simulink library "outp"  (R2021b)
(part 3 of 11)

  outpmodule/365(VOUTP_C3CCU1CSDTC_raw32) -> bus_creator/365
  bus_selector17/58 -> outpmodule/1117(VVMC_ADASWarningMsg_enum)  "<VVMC_ADASWarningMsg_enum>"
  bus_selector13/20 -> outpmodule/907(VTPM_RRWheelDebug_flg)  "<VTPM_RRWheelDebug_flg>"
  bus_selector17/62 -> outpmodule/1121(VVMC_LKAHODDisplayWarning_flg)  "<VVMC_LKAHODDisplayWarning_flg>"
  bus_selector17/53 -> outpmodule/1112(VVMC_ADASLDWSta_enum)  "<VVMC_ADASLDWSta_enum>"
  bus_selector17/50 -> outpmodule/1109(VVMC_RightTurnLightReq_flg)  "<VVMC_RightTurnLightReq_flg>"
  bus_selector17/47 -> outpmodule/1106(VVMC_ADASShftPosnReq_enum)  "<VVMC_ADASShftPosnReq_enum>"
  bus_selector17/46 -> outpmodule/1105(VVMC_ADASShftPosnReqA_flg)  "<VVMC_ADASShftPosnReqA_flg>"
  outpmodule/566(VOUTP_KeyAreaSPTGSta_enum) -> bus_creator/566
  bus_selector4/65 -> outpmodule/422(VDDM_FMLUSSDTC_raw32)  "<VDDM_FMLUSSDTC_raw32>"
  bus_selector9/3 -> outpmodule/611(VNMM_Awake_enum)  "<VNMM_Awake_enum>"
  outpmodule/81(VOUTP_RFPulseCount_enum) -> bus_creator/81
  outpmodule/479(VOUTP_RRWheelTmpHighDTC_raw32) -> bus_creator/479
  outpmodule/291(VOUTP_DimSwSta_flg) -> bus_creator/291
  bus_selector17/43 -> outpmodule/1102(VVMC_ACCJerkLowerLimit_mps3)  "<VVMC_ACCJerkLowerLimit_mps3>"
  bus_selector13/8 -> outpmodule/895(VTPM_RRWheelPress_raw8)  "<VTPM_RRWheelPress_raw8>"
  bus_selector2/60 -> outpmodule/63(VAPM_LFWhlRotDir_enum)  "<VAPM_LFWhlRotDir_enum>"
  bus_selector17/42 -> outpmodule/1101(VVMC_ACCComfortBandUpper_mps2)  "<VVMC_ACCComfortBandUpper_mps2>"
  outpmodule/551(VOUTP_PKELNumerator_kphsqr) -> bus_creator/551
  bus_selector7/47 -> outpmodule/601(VDKC_UWBDetArea_enum)  "<VDKC_UWBDetArea_enum>"
  bus_selector17/36 -> outpmodule/1095(VVMC_ADASDBSReq_enum)  "<VVMC_ADASDBSReq_enum>"
  bus_selector17/34 -> outpmodule/1093(VVMC_AEBVehHoldReq_flg)  "<VVMC_AEBVehHoldReq_flg>"
  bus_selector17/35 -> outpmodule/1094(VVMC_ACCVehHoldReq_flg)  "<VVMC_ACCVehHoldReq_flg>"
  bus_selector17/31 -> outpmodule/1090(VVMC_LKATOIAct_enum)  "<VVMC_LKATOIAct_enum>"
  outpmodule/556(VOUTP_DKCAuthSta_enum) -> bus_creator/556
  bus_selector17/32 -> outpmodule/1091(VVMC_ADASAEBReq_enum)  "<VVMC_ADASAEBReq_enum>"
  outpmodule/1063(VOUTP_MeterIndSpeed_raw32) -> bus_creator/1063
  bus_selector17/28 -> outpmodule/1087(VVMC_ADASLKASta_enum)  "<VVMC_ADASLKASta_enum>"
  bus_selector17/26 -> outpmodule/1085(VVMC_ActACCRequiredAccel_mps2)  "<VVMC_ActACCRequiredAccel_mps2>"
  bus_selector13/2 -> outpmodule/889(VTPM_RFBatWarn_flg)  "<VTPM_RFBatWarn_flg>"
  outpmodule/221(VOUTP_FrWiperL_flg) -> bus_creator/221
  bus_selector17/27 -> outpmodule/1086(VVMC_LateralCtrl_flg)  "<VVMC_LateralCtrl_flg>"
  bus_selector3/106 -> outpmodule/284(VBCM_AmbBrightnessSta1_enum)  "<VBCM_AmbBrightnessSta1_enum>"
  outpmodule/276(VOUTP_AmbPwrWarnENFlash_enum) -> bus_creator/276
  bus_selector2/38 -> outpmodule/41(VAPM_Chime_enum)  "<VAPM_Chime_enum>"
  bus_selector17/24 -> outpmodule/1083(VVMC_DISCReqAcc_mps2)  "<VVMC_DISCReqAcc_mps2>"
  bus_selector17/23 -> outpmodule/1082(VVMC_ACCRequiredAccel_mps2)  "<VVMC_ACCRequiredAccel_mps2>"
  bus_selector17/22 -> outpmodule/1081(VVMC_ISOJerkLimit_mps3)  "<VVMC_ISOJerkLimit_mps3>"
  bus_selector17/19 -> outpmodule/1078(VVMC_AccCalcuPID_mps2)  "<VVMC_AccCalcuPID_mps2>"
  outpmodule/450(VOUTP_ACCMalfuncDetDTC_raw32) -> bus_creator/450
  bus_selector17/18 -> outpmodule/1077(VVMC_SPD2ACCAct_flg)  "<VVMC_SPD2ACCAct_flg>"
  bus_selector12/17 -> outpmodule/728(VTHC_FDFrRiAPTCHeatPwrCmd_W)  "<VTHC_FDFrRiAPTCHeatPwrCmd_W>"
  outpmodule/1088(VOUTP_LKAStrToqReq_Nm) -> bus_creator/1088
  outpmodule/518(VOUTP_LowIdleAccPedal_flg) -> bus_creator/518
  outpmodule/909(VOUTP_TPMSCaliButtAllow_flg) -> bus_creator/909
  bus_selector7/48 -> outpmodule/602(VDKC_OutputPCMDModule_enum)  "<VDKC_OutputPCMDModule_enum>"
  outpmodule/415(VOUTP_EnterNewOperCyc_flg) -> bus_creator/415
  bus_selector12/16 -> outpmodule/727(VTHC_FDFrLeAPTCHeatPwrCmd_W)  "<VTHC_FDFrLeAPTCHeatPwrCmd_W>"
  bus_selector12/14 -> outpmodule/725(VTHC_FDEWP2Cmd_enum)  "<VTHC_FDEWP2Cmd_enum>"
  outpmodule/410(VOUTP_MCUR1NoComDTC_raw32) -> bus_creator/410
  bus_selector17/60 -> outpmodule/1119(VVMC_TargetType_enum)  "<VVMC_TargetType_enum>"
  outpmodule/278(VOUTP_AmbColorSta1_enum) -> bus_creator/278
  bus_selector12/15 -> outpmodule/726(VTHC_FDEWP3Cmd_enum)  "<VTHC_FDEWP3Cmd_enum>"
  bus_selector12/12 -> outpmodule/723(VTHC_FDAGSCmd_enum)  "<VTHC_FDAGSCmd_enum>"
  outpmodule/938(VOUTP_LFP20_raw8) -> bus_creator/938
  outpmodule/944(VOUTP_S1WheelDebugALTU_pct) -> bus_creator/944
  bus_selector12/13 -> outpmodule/724(VTHC_FDEWP1Cmd_enum)  "<VTHC_FDEWP1Cmd_enum>"
  bus_selector12/11 -> outpmodule/722(VTHC_CoolgFanActDuty_pct)  "<VTHC_CoolgFanActDuty_pct>"
  bus_selector12/9 -> outpmodule/720(VTHC_FDTWVCmd_pct)  "<VTHC_FDTWVCmd_pct>"
  outpmodule/137(VOUTP_AVMparkingcancel_enum) -> bus_creator/137
  outpmodule/929(VOUTP_S1ID_raw32) -> bus_creator/929
  bus_selector7/8 -> outpmodule/562(VDKC_KeyNumSta_enum)  "<VDKC_KeyNumSta_enum>"
  bus_selector3/43 -> outpmodule/221(VBCM_FrWiperL_flg)  "<VBCM_FrWiperL_flg>"
  outpmodule/886(VOUTP_FDCFGSFuncSta_flg) -> bus_creator/886
  bus_selector12/10 -> outpmodule/721(VTHC_FDFrWPTCHeatPwrCmd_W)  "<VTHC_FDFrWPTCHeatPwrCmd_W>"
  bus_selector12/6 -> outpmodule/717(VTHC_FDEXV2Cmd_step)  "<VTHC_FDEXV2Cmd_step>"
  outpmodule/100(VOUTP_SASCALTimeOut_flg) -> bus_creator/100
  bus_selector7/29 -> outpmodule/583(VDKC_UWBDetPTGArea_enum)  "<VDKC_UWBDetPTGArea_enum>"
  outpmodule/198(VOUTP_Dimmer_pct) -> bus_creator/198
  outpmodule/361(VOUTP_C3BMS1RCDTC_raw32) -> bus_creator/361
  outpmodule/223(VOUTP_RrWiper_flg) -> bus_creator/223
  bus_selector12/7 -> outpmodule/718(VTHC_FDSOTXVCmd_flg)  "<VTHC_FDSOTXVCmd_flg>"
  bus_selector17/2 -> outpmodule/1061(VVMC_VehicleSpeed_mph)  "<VVMC_VehicleSpeed_mph>"
  outpmodule/585(VOUTP_ParkingModeCmd_enum) -> bus_creator/585
  bus_selector2/100 -> outpmodule/103(VAPM_GRADE_Deg)  "<VAPM_GRADE_Deg>"
  bus_selector12/4 -> outpmodule/715(VTHC_FDSOV3Cmd_flg)  "<VTHC_FDSOV3Cmd_flg>"
  bus_selector12/2 -> outpmodule/713(VTHC_FDSOV1Cmd_flg)  "<VTHC_FDSOV1Cmd_flg>"
  bus_selector2/103 -> outpmodule/106(VAPM_YawRateTimeOut_flg)  "<VAPM_YawRateTimeOut_flg>"
  outpmodule/72(VOUTP_LFPulseCountVTimeOut_flg) -> bus_creator/72
  bus_selector12/97 -> outpmodule/808(VTHC_AirIntenZone3MSet7_enum)  "<VTHC_AirIntenZone3MSet7_enum>"
  bus_selector12/3 -> outpmodule/714(VTHC_FDSOV2Cmd_flg)  "<VTHC_FDSOV2Cmd_flg>"
  outpmodule/690(VOUTP_SHA1_cnt) -> bus_creator/690
  outpmodule/134(VOUTP_EPBErrStaTimeOut_flg) -> bus_creator/134
  bus_selector3/75 -> outpmodule/253(VBCM_MFRDNBrightReq_pct)  "<VBCM_MFRDNBrightReq_pct>"
  bus_selector11/17 -> outpmodule/685(VSYS_Variation_cnt)  "<VSYS_Variation_cnt>"
  bus_selector14/46 -> outpmodule/1030(VTQD_OPDHoldLamp_flg)  "<VTQD_OPDHoldLamp_flg>"
  bus_selector11/15 -> outpmodule/683(VSYS_Country1_cnt)  "<VSYS_Country1_cnt>"
  bus_selector7/12 -> outpmodule/566(VDKC_KeyAreaSPTGSta_enum)  "<VDKC_KeyAreaSPTGSta_enum>"
  bus_selector11/12 -> outpmodule/680(VSYS_Minor2_cnt)  "<VSYS_Minor2_cnt>"
  bus_selector13/9 -> outpmodule/896(VTPM_LFWheelTemp_C)  "<VTPM_LFWheelTemp_C>"
  outpmodule/629(VOUTP_HVSysReadyToCharge_enum) -> bus_creator/629
  bus_selector3/138 -> outpmodule/316(VBCM_WelcomeLight_enum)  "<VBCM_WelcomeLight_enum>"
  bus_selector11/10 -> outpmodule/678(VSYS_Major2_cnt)  "<VSYS_Major2_cnt>"
  outpmodule/774(VOUTP_FDCTHCCLVentENSta_flg) -> bus_creator/774
  bus_selector11/6 -> outpmodule/674(VSYS_CarModel3_cnt)  "<VSYS_CarModel3_cnt>"
  bus_selector11/5 -> outpmodule/673(VSYS_CarModel2_cnt)  "<VSYS_CarModel2_cnt>"
  outpmodule/215(VOUTP_MirrorDefog_flg) -> bus_creator/215
  outpmodule/315(VOUTP_HoodRelCmd_flg) -> bus_creator/315
  bus_selector17/49 -> outpmodule/1108(VVMC_HazardWarningReq_flg)  "<VVMC_HazardWarningReq_flg>"
  bus_selector11/3 -> outpmodule/671(VSYS_HWVer3_cnt)  "<VSYS_HWVer3_cnt>"
  outpmodule/1035(VOUTP_SetSpd_kph) -> bus_creator/1035
  bus_selector13/64 -> outpmodule/951(VTPM_ID4messageALTU_raw8)  "<VTPM_ID4messageALTU_raw8>"
  bus_selector12/18 -> outpmodule/729(VTHC_FDRrAPTCHeatPwrCmd_W)  "<VTHC_FDRrAPTCHeatPwrCmd_W>"
  outpmodule/1124(VOUTP_ADASLaneModeL_enum) -> bus_creator/1124
  bus_selector11/4 -> outpmodule/672(VSYS_CarModel1_cnt)  "<VSYS_CarModel1_cnt>"
  outpmodule/419(VOUTP_DiagRLTSDTC_raw32) -> bus_creator/419
  bus_selector11/1 -> outpmodule/669(VSYS_HWVer1_cnt)  "<VSYS_HWVer1_cnt>"
  BPMM_outputs/1 -> bus_selector10/1
  bus_selector10/47 -> outpmodule/667(VPMM_OTAPwrReqStdChkSta_enum)  "<VPMM_OTAPwrReqStdChkSta_enum>"
  outpmodule/115(VOUTP_LatAccelV_flg) -> bus_creator/115
  bus_selector13/41 -> outpmodule/928(VTPM_RRSensorMode_flg)  "<VTPM_RRSensorMode_flg>"
  outpmodule/839(VOUTP_FDCTHCREVentZStaSet7_enum) -> bus_creator/839
  bus_selector10/46 -> outpmodule/666(VPMM_OTAPwrReqOFFChkSta_enum)  "<VPMM_OTAPwrReqOFFChkSta_enum>"
  bus_selector3/123 -> outpmodule/301(VBCM_TurnSwTimeSetSta457_enum)  "<VBCM_TurnSwTimeSetSta457_enum>"
  bus_selector10/48 -> outpmodule/668(VPMM_PwrReqRAPSAvail_flg)  "<VPMM_PwrReqRAPSAvail_flg>"
  bus_selector12/105 -> outpmodule/816(VTHC_RVentENSet_enum)  "<VTHC_RVentENSet_enum>"
  bus_selector2/136 -> outpmodule/139(VAPM_AVMparkingexcute_enum)  "<VAPM_AVMparkingexcute_enum>"
  bus_selector10/44 -> outpmodule/664(VPMM_Sched_ChgTOSta_enum)  "<VPMM_Sched_ChgTOSta_enum>"
  bus_selector4/147 -> outpmodule/504(VDDM_SysAllowReadySta_flg)  "<VDDM_SysAllowReadySta_flg>"
  bus_selector7/26 -> outpmodule/580(VDKC_AllowSleep_flg)  "<VDKC_AllowSleep_flg>"
  bus_selector14/43 -> outpmodule/1027(VTQD_ActParkRequest_flg)  "<VTQD_ActParkRequest_flg>"
  bus_selector10/45 -> outpmodule/665(VPMM_PwrReq_OTA_enum)  "<VPMM_PwrReq_OTA_enum>"
  bus_selector3/30 -> outpmodule/208(VBCM_LBSD_flg)  "<VBCM_LBSD_flg>"
  bus_selector4/121 -> outpmodule/478(VDDM_LRWheelTmpHighDTC_raw32)  "<VDDM_LRWheelTmpHighDTC_raw32>"
  outpmodule/508(VOUTP_CAN2BusErrorDTC_raw32) -> bus_creator/508
  bus_selector12/69 -> outpmodule/780(VTHC_FDCFGSAirIntSta_enum)  "<VTHC_FDCFGSAirIntSta_enum>"
  bus_selector12/68 -> outpmodule/779(VTHC_FDCTHCMAPTCForceOFFSta_flg)  "<VTHC_FDCTHCMAPTCForceOFFSta_flg>"
  bus_selector1/1 -> outpmodule/1(VACC_HVTHCMSysAvail_enum)  "<VACC_HVTHCMSysAvail_enum>"
  bus_selector12/64 -> outpmodule/775(VTHC_FDCTHCREVentYSta_enum)  "<VTHC_FDCTHCREVentYSta_enum>"
  bus_selector12/67 -> outpmodule/778(VTHC_FDCTHCCRVentENSta_flg)  "<VTHC_FDCTHCCRVentENSta_flg>"
  outpmodule/120(VOUTP_MCPressureVTimeOut_flg) -> bus_creator/120
  outpmodule/238(VOUTP_AmbLightColor1_enum) -> bus_creator/238
  bus_selector12/65 -> outpmodule/776(VTHC_FDCTHCRVentENSta_flg)  "<VTHC_FDCTHCRVentENSta_flg>"
  outpmodule/93(VOUTP_SASAngle_Deg) -> bus_creator/93
  bus_selector12/62 -> outpmodule/773(VTHC_FDCTHCCLEVentYSta_enum)  "<VTHC_FDCTHCCLEVentYSta_enum>"
  bus_selector12/61 -> outpmodule/772(VTHC_FDCTHCLVentENSta_flg)  "<VTHC_FDCTHCLVentENSta_flg>"
  bus_selector12/60 -> outpmodule/771(VTHC_FDCTHCLEVentYSta_enum)  "<VTHC_FDCTHCLEVentYSta_enum>"
  outpmodule/454(VOUTP_MCUF1RCErrDTC_raw32) -> bus_creator/454
  outpmodule/874(VOUTP_SettempZon1Set5_enum) -> bus_creator/874
  outpmodule/888(VOUTP_LFBatWarn_flg) -> bus_creator/888
  bus_selector12/59 -> outpmodule/770(VTHC_FDCTHCCREVentZSta_enum)  "<VTHC_FDCTHCCREVentZSta_enum>"
  bus_selector2/51 -> outpmodule/54(VAPM_RRRawWhlSpeedTimeOut_flg)  "<VAPM_RRRawWhlSpeedTimeOut_flg>"
  bus_selector12/55 -> outpmodule/766(VTHC_FDCTHCREVentModeSta_enum)  "<VTHC_FDCTHCREVentModeSta_enum>"
  bus_selector12/57 -> outpmodule/768(VTHC_FDCTHCCLEVentZSta_enum)  "<VTHC_FDCTHCCLEVentZSta_enum>"
  outpmodule/659(VOUTP_CtrlFrBMSCCUCIR_flg) -> bus_creator/659
  bus_selector12/53 -> outpmodule/764(VTHC_FDCTHCAirIntZ3Sta_enum)  "<VTHC_FDCTHCAirIntZ3Sta_enum>"
  bus_selector4/59 -> outpmodule/416(VDDM_DiagHCrashDTC_raw32)  "<VDDM_DiagHCrashDTC_raw32>"
  BACC_outputs/1 -> bus_selector1/1
  outpmodule/90(VOUTP_DriIntendTimeOut_flg) -> bus_creator/90
  bus_selector7/40 -> outpmodule/594(VDKC_BLERSSI_enum)  "<VDKC_BLERSSI_enum>"
  bus_selector12/52 -> outpmodule/763(VTHC_sigDfrstSt_flg)  "<VTHC_sigDfrstSt_flg>"
  bus_selector12/50 -> outpmodule/761(VTHC_fdefog_flg)  "<VTHC_fdefog_flg>"
  bus_selector12/48 -> outpmodule/759(VTHC_RecAutoFlg_flg)  "<VTHC_RecAutoFlg_flg>"
  bus_selector2/22 -> outpmodule/25(VAPM_PASARCL_enum)  "<VAPM_PASARCL_enum>"
  bus_selector11/2 -> outpmodule/670(VSYS_HWVer2_cnt)  "<VSYS_HWVer2_cnt>"
  outpmodule/122(VOUTP_BrkSwStaTimeOut_flg) -> bus_creator/122
  bus_selector12/46 -> outpmodule/757(VTHC_CCUSyncSts_flg)  "<VTHC_CCUSyncSts_flg>"
  outpmodule/126(VOUTP_ESCStandstillTimeOut_flg) -> bus_creator/126
  outpmodule/882(VOUTP_CLVentEN_flg) -> bus_creator/882
  bus_selector9/5 -> outpmodule/613(VNMM_ErrorState_enum)  "<VNMM_ErrorState_enum>"
  outpmodule/214(VOUTP_MirrorCtrl_enum) -> bus_creator/214
  outpmodule/577(VOUTP_FDCSPTGOpen_flg) -> bus_creator/577
  bus_selector2/82 -> outpmodule/85(VAPM_RRPulseCount_enum)  "<VAPM_RRPulseCount_enum>"
  bus_selector3/2 -> outpmodule/180(VBCM_TailgateRemote_enum)  "<VBCM_TailgateRemote_enum>"
  outpmodule/1171(VOUTP_FDCVMCAPSRqEPSCtrl_flg) -> bus_creator/1171
  bus_selector12/63 -> outpmodule/774(VTHC_FDCTHCCLVentENSta_flg)  "<VTHC_FDCTHCCLVentENSta_flg>"
  bus_selector12/44 -> outpmodule/755(VTHC_FaceM_flg)  "<VTHC_FaceM_flg>"
  outpmodule/11(VOUTP_PASDRCR_cm) -> bus_creator/11
  bus_selector12/45 -> outpmodule/756(VTHC_FootM_flg)  "<VTHC_FootM_flg>"
  outpmodule/128(VOUTP_ESCAPSStaTimeOut_flg) -> bus_creator/128
  bus_selector2/104 -> outpmodule/107(VAPM_LatAccel_Gps)  "<VAPM_LatAccel_Gps>"
  bus_selector12/42 -> outpmodule/753(VTHC_Foot_flg)  "<VTHC_Foot_flg>"
  bus_selector2/144 -> outpmodule/147(VAPM_CAASSw_enum)  "<VAPM_CAASSw_enum>"
  outpmodule/780(VOUTP_FDCFGSAirIntSta_enum) -> bus_creator/780
  outpmodule/530(VOUTP_APPD_pct) -> bus_creator/530
  bus_selector7/35 -> outpmodule/589(VDKC_DKeyWelcomeSta_enum)  "<VDKC_DKeyWelcomeSta_enum>"
  bus_selector12/39 -> outpmodule/750(VTHC_FDRecyAutoCmd_enum)  "<VTHC_FDRecyAutoCmd_enum>"
  bus_selector2/93 -> outpmodule/96(VAPM_SASSpeedTimeOut_flg)  "<VAPM_SASSpeedTimeOut_flg>"
  outpmodule/96(VOUTP_SASSpeedTimeOut_flg) -> bus_creator/96
  bus_selector12/43 -> outpmodule/754(VTHC_Frost_flg)  "<VTHC_Frost_flg>"
  outpmodule/707(VOUTP_PmicBootPath_raw32) -> bus_creator/707
  bus_selector17/63 -> outpmodule/1122(VVMC_LKAHODSoundWarning_flg)  "<VVMC_LKAHODSoundWarning_flg>"
  bus_selector2/16 -> outpmodule/19(VAPM_APSDFLR_cm)  "<VAPM_APSDFLR_cm>"
  bus_selector12/41 -> outpmodule/752(VTHC_Face_flg)  "<VTHC_Face_flg>"
  bus_selector2/156 -> outpmodule/159(VAPM_APSSWVer_enum)  "<VAPM_APSSWVer_enum>"
  bus_selector12/34 -> outpmodule/745(VTHC_sigClntTHvBattIn_C)  "<VTHC_sigClntTHvBattIn_C>"
  bus_selector12/36 -> outpmodule/747(VTHC_sigAmbAirT_C)  "<VTHC_sigAmbAirT_C>"
  bus_selector17/21 -> outpmodule/1080(VVMC_ISODecLimit_mps2)  "<VVMC_ISODecLimit_mps2>"
  bus_selector11/8 -> outpmodule/676(VSYS_ECU2_cnt)  "<VSYS_ECU2_cnt>"
  bus_selector12/33 -> outpmodule/744(VTHC_sigCbnSolarLeft_W)  "<VTHC_sigCbnSolarLeft_W>"
  bus_selector12/32 -> outpmodule/743(VTHC_sigClntTHvBattOut_C)  "<VTHC_sigClntTHvBattOut_C>"
  outpmodule/294(VOUTP_FWasSwSta_enum) -> bus_creator/294
  outpmodule/83(VOUTP_LRPulseCount_enum) -> bus_creator/83
  bus_selector12/29 -> outpmodule/740(VTHC_sigRecircSt_flg)  "<VTHC_sigRecircSt_flg>"
  bus_selector12/31 -> outpmodule/742(VTHC_sigSetTempZon2St_C)  "<VTHC_sigSetTempZon2St_C>"
  bus_selector12/28 -> outpmodule/739(VTHC_sigWindDirZon1St_enum)  "<VTHC_sigWindDirZon1St_enum>"
  bus_selector3/98 -> outpmodule/276(VBCM_AmbPwrWarnENFlash_enum)  "<VBCM_AmbPwrWarnENFlash_enum>"
  bus_selector17/105 -> outpmodule/1164(VVMC_CalibratedAccY_G)  "<VVMC_CalibratedAccY_G>"
  bus_selector4/23 -> outpmodule/380(VDDM_ONtoRdyDTC_raw32)  "<VDDM_ONtoRdyDTC_raw32>"
  bus_selector10/29 -> outpmodule/649(VPMM_LVBattChrgTimeCnt_s)  "<VPMM_LVBattChrgTimeCnt_s>"
  outpmodule/108(VOUTP_LatAccelTimeOut_flg) -> bus_creator/108
  bus_selector12/27 -> outpmodule/738(VTHC_sigAirIntenZon1St_enum)  "<VTHC_sigAirIntenZon1St_enum>"
  bus_selector3/57 -> outpmodule/235(VBCM_AmbLightBrightness4_enum)  "<VBCM_AmbLightBrightness4_enum>"
  outpmodule/919(VOUTP_LFWheelPSW_raw8) -> bus_creator/919
  bus_selector13/32 -> outpmodule/919(VTPM_LFWheelPSW_raw8)  "<VTPM_LFWheelPSW_raw8>"
  outpmodule/734(VOUTP_CCUACLampSts_flg) -> bus_creator/734
  bus_selector12/25 -> outpmodule/736(VTHC_CCUACMaxLampSts_flg)  "<VTHC_CCUACMaxLampSts_flg>"
  bus_selector12/22 -> outpmodule/733(VTHC_CabinMode_enum)  "<VTHC_CabinMode_enum>"
  outpmodule/412(VOUTP_ESC7NoComDTC_raw32) -> bus_creator/412
  bus_selector12/167 -> outpmodule/878(VTHC_FACESet_enum)  "<VTHC_FACESet_enum>"
  bus_selector12/166 -> outpmodule/877(VTHC_ACModeSet457_enum)  "<VTHC_ACModeSet457_enum>"
  outpmodule/935(VOUTP_S3L_enum) -> bus_creator/935
  bus_selector4/41 -> outpmodule/398(VDDM_FLDoorSWDTC_raw32)  "<VDDM_FLDoorSWDTC_raw32>"
  bus_selector12/168 -> outpmodule/879(VTHC_FOOTSet_enum)  "<VTHC_FOOTSet_enum>"
  bus_selector12/164 -> outpmodule/875(VTHC_SettempZon1Set7_enum)  "<VTHC_SettempZon1Set7_enum>"
  bus_selector4/9 -> outpmodule/366(VDDM_C3CCU1LCDTC_raw32)  "<VDDM_C3CCU1LCDTC_raw32>"
  bus_selector12/8 -> outpmodule/719(VTHC_FDFWVCmd_flg)  "<VTHC_FDFWVCmd_flg>"
  bus_selector17/48 -> outpmodule/1107(VVMC_ADASForceIdle_flg)  "<VVMC_ADASForceIdle_flg>"
  bus_selector17/29 -> outpmodule/1088(VVMC_LKAStrToqReq_Nm)  "<VVMC_LKAStrToqReq_Nm>"
  outpmodule/590(VOUTP_UWB1Distance_enum) -> bus_creator/590
  bus_selector12/162 -> outpmodule/873(VTHC_SettempZon1Set4_enum)  "<VTHC_SettempZon1Set4_enum>"
  bus_selector12/163 -> outpmodule/874(VTHC_SettempZon1Set5_enum)  "<VTHC_SettempZon1Set5_enum>"
  bus_selector17/38 -> outpmodule/1097(VVMC_ACCObjDist_m)  "<VVMC_ACCObjDist_m>"
  bus_selector7/38 -> outpmodule/592(VDKC_UWB3Distance_enum)  "<VDKC_UWB3Distance_enum>"
  bus_selector12/161 -> outpmodule/872(VTHC_SettempZon1Set3_enum)  "<VTHC_SettempZon1Set3_enum>"
  bus_selector12/159 -> outpmodule/870(VTHC_SettempZon1Set1_enum)  "<VTHC_SettempZon1Set1_enum>"
  outpmodule/738(VOUTP_sigAirIntenZon1St_enum) -> bus_creator/738
  bus_selector17/65 -> outpmodule/1124(VVMC_ADASLaneModeL_enum)  "<VVMC_ADASLaneModeL_enum>"
  bus_selector12/158 -> outpmodule/869(VTHC_FDCTHCCREVentYStaSet7_enum)  "<VTHC_FDCTHCCREVentYStaSet7_enum>"
  outpmodule/1163(VOUTP_CalibratedAccX_G) -> bus_creator/1163
  bus_selector3/24 -> outpmodule/202(VBCM_HBeam_flg)  "<VBCM_HBeam_flg>"
  bus_selector13/37 -> outpmodule/924(VTPM_AutoLTips_enum)  "<VTPM_AutoLTips_enum>"
  bus_selector17/37 -> outpmodule/1096(VVMC_ADASACCSta_enum)  "<VVMC_ADASACCSta_enum>"
  bus_selector12/155 -> outpmodule/866(VTHC_FDCTHCCREVentYStaSet3_enum)  "<VTHC_FDCTHCCREVentYStaSet3_enum>"
  bus_selector3/69 -> outpmodule/247(VBCM_FollowMe_flg)  "<VBCM_FollowMe_flg>"
  outpmodule/601(VOUTP_UWBDetArea_enum) -> bus_creator/601
  outpmodule/49(VOUTP_RFRawWhlSpeed_kph) -> bus_creator/49
  bus_selector12/151 -> outpmodule/862(VTHC_FDCTHCREVentYStaSet5_enum)  "<VTHC_FDCTHCREVentYStaSet5_enum>"
  bus_selector13/44 -> outpmodule/931(VTPM_S3ID_raw32)  "<VTPM_S3ID_raw32>"
  bus_selector4/18 -> outpmodule/375(VDDM_Lv3ErrDTC_raw32)  "<VDDM_Lv3ErrDTC_raw32>"
  outpmodule/438(VOUTP_FCM3CSErrDTC_raw32) -> bus_creator/438
  bus_selector17/40 -> outpmodule/1099(VVMC_TimeGapLevel_enum)  "<VVMC_TimeGapLevel_enum>"
  bus_selector12/153 -> outpmodule/864(VTHC_FDCTHCCREVentYStaSet1_enum)  "<VTHC_FDCTHCCREVentYStaSet1_enum>"
  outpmodule/51(VOUTP_LRRawWhlSpeed_kph) -> bus_creator/51
  bus_selector13/4 -> outpmodule/891(VTPM_RRBatWarn_flg)  "<VTPM_RRBatWarn_flg>"
  bus_selector4/53 -> outpmodule/410(VDDM_MCUR1NoComDTC_raw32)  "<VDDM_MCUR1NoComDTC_raw32>"
  outpmodule/655(VOUTP_LVSilentChrgReq_flg) -> bus_creator/655
  bus_selector12/154 -> outpmodule/865(VTHC_FDCTHCCREVentYStaSet2_enum)  "<VTHC_FDCTHCCREVentYStaSet2_enum>"
  bus_selector10/27 -> outpmodule/647(VPMM_IVIPwrStaONTOPopT_s)  "<VPMM_IVIPwrStaONTOPopT_s>"
  bus_selector12/149 -> outpmodule/860(VTHC_FDCTHCREVentYStaSet3_enum)  "<VTHC_FDCTHCREVentYStaSet3_enum>"
  bus_selector11/13 -> outpmodule/681(VSYS_Patch1_cnt)  "<VSYS_Patch1_cnt>"
  bus_selector4/83 -> outpmodule/440(VDDM_FCM4CSErrDTC_raw32)  "<VDDM_FCM4CSErrDTC_raw32>"
  outpmodule/453(VOUTP_ISAMalfuncDetDTC_raw32) -> bus_creator/453
  bus_selector12/150 -> outpmodule/861(VTHC_FDCTHCREVentYStaSet4_enum)  "<VTHC_FDCTHCREVentYStaSet4_enum>"
  outpmodule/300(VOUTP_TurnSwTimeSetSta123_enum) -> bus_creator/300
  bus_selector12/54 -> outpmodule/765(VTHC_FDCTHCLEVentModeSta_enum)  "<VTHC_FDCTHCLEVentModeSta_enum>"
  bus_selector12/146 -> outpmodule/857(VTHC_FDCTHCCLEVentYStaSet7_enum)  "<VTHC_FDCTHCCLEVentYStaSet7_enum>"
  bus_selector12/148 -> outpmodule/859(VTHC_FDCTHCREVentYStaSet2_enum)  "<VTHC_FDCTHCREVentYStaSet2_enum>"
  outpmodule/705(VOUTP_ECUGen1_cnt) -> bus_creator/705
  outpmodule/1045(VOUTP_FrTMTqReq_Nm) -> bus_creator/1045
  bus_selector17/41 -> outpmodule/1100(VVMC_ACCJerkUpperLimit_mps3)  "<VVMC_ACCJerkUpperLimit_mps3>"
  bus_selector12/147 -> outpmodule/858(VTHC_FDCTHCREVentYStaSet1_enum)  "<VTHC_FDCTHCREVentYStaSet1_enum>"
  bus_selector12/143 -> outpmodule/854(VTHC_FDCTHCCLEVentYStaSet3_enum)  "<VTHC_FDCTHCCLEVentYStaSet3_enum>"
  bus_selector4/72 -> outpmodule/429(VDDM_FLLUSSDTC_raw32)  "<VDDM_FLLUSSDTC_raw32>"
  bus_selector12/145 -> outpmodule/856(VTHC_FDCTHCCLEVentYStaSet5_enum)  "<VTHC_FDCTHCCLEVentYStaSet5_enum>"
  bus_selector12/141 -> outpmodule/852(VTHC_FDCTHCCLEVentYStaSet1_enum)  "<VTHC_FDCTHCCLEVentYStaSet1_enum>"
  bus_selector6/3 -> outpmodule/528(VDID_MILDIST_km)  "<VDID_MILDIST_km>"
  bus_selector11/11 -> outpmodule/679(VSYS_Minor1_cnt)  "<VSYS_Minor1_cnt>"
  outpmodule/1103(VOUTP_ACCComfortBandLower_mps2) -> bus_creator/1103
  bus_selector12/138 -> outpmodule/849(VTHC_FDCTHCLEVentYStaSet4_enum)  "<VTHC_FDCTHCLEVentYStaSet4_enum>"
  bus_selector17/52 -> outpmodule/1111(VVMC_ADASFCWSta_enum)  "<VVMC_ADASFCWSta_enum>"
  outpmodule/550(VOUTP_PKERNumerator_kphsqr) -> bus_creator/550
  bus_selector17/57 -> outpmodule/1116(VVMC_ACCTakeoverReq_flg)  "<VVMC_ACCTakeoverReq_flg>"
  bus_selector13/77 -> outpmodule/964(VTPM_WriteChkRRID_raw)  "<VTPM_WriteChkRRID_raw>"
  bus_selector4/81 -> outpmodule/438(VDDM_FCM3CSErrDTC_raw32)  "<VDDM_FCM3CSErrDTC_raw32>"
  bus_selector2/168 -> outpmodule/171(VAPM_APSSpeedCMD_kph)  "<VAPM_APSSpeedCMD_kph>"
  bus_selector9/4 -> outpmodule/612(VNMM_CSB_flg)  "<VNMM_CSB_flg>"
  bus_selector12/139 -> outpmodule/850(VTHC_FDCTHCLEVentYStaSet5_enum)  "<VTHC_FDCTHCLEVentYStaSet5_enum>"
  bus_selector4/156 -> outpmodule/513(VDDM_FrMCU4PreDTC_raw32)  "<VDDM_FrMCU4PreDTC_raw32>"
  outpmodule/686(VOUTP_Dash1_cnt) -> bus_creator/686
  outpmodule/287(VOUTP_AmbBrightnessSta4_enum) -> bus_creator/287
  bus_selector7/24 -> outpmodule/578(VDKC_UIDLowPowerSta_flg)  "<VDKC_UIDLowPowerSta_flg>"
  bus_selector2/3 -> outpmodule/6(VAPM_FSOffSw_enum)  "<VAPM_FSOffSw_enum>"
  bus_selector12/135 -> outpmodule/846(VTHC_FDCTHCLEVentYStaSet1_enum)  "<VTHC_FDCTHCLEVentYStaSet1_enum>"
  bus_selector3/97 -> outpmodule/275(VBCM_AmbLinkDriStaFlash_enum)  "<VBCM_AmbLinkDriStaFlash_enum>"
  bus_selector12/137 -> outpmodule/848(VTHC_FDCTHCLEVentYStaSet3_enum)  "<VTHC_FDCTHCLEVentYStaSet3_enum>"
  outpmodule/94(VOUTP_SASAngleTimeOut_flg) -> bus_creator/94
  outpmodule/505(VOUTP_VCUHoodSWSta_flg) -> bus_creator/505
  bus_selector13/52 -> outpmodule/939(VTPM_RFP20_raw8)  "<VTPM_RFP20_raw8>"
  outpmodule/670(VOUTP_HWVer2_cnt) -> bus_creator/670
  bus_selector17/55 -> outpmodule/1114(VVMC_ACCObjDstLvl_enum)  "<VVMC_ACCObjDstLvl_enum>"
  outpmodule/360(VOUTP_C3BMS6LCDTC_raw32) -> bus_creator/360
  bus_selector12/136 -> outpmodule/847(VTHC_FDCTHCLEVentYStaSet2_enum)  "<VTHC_FDCTHCLEVentYStaSet2_enum>"
  outpmodule/703(VOUTP_AcoreRebootCmdACK_flg) -> bus_creator/703
  bus_selector12/132 -> outpmodule/843(VTHC_FDCTHCCREVentZStaSet4_enum)  "<VTHC_FDCTHCCREVentZStaSet4_enum>"
  bus_selector7/15 -> outpmodule/569(VDKC_UWBOnOff_flg)  "<VDKC_UWBOnOff_flg>"
  outpmodule/538(VOUTP_CPSAR_sec) -> bus_creator/538
  bus_selector17/44 -> outpmodule/1103(VVMC_ACCComfortBandLower_mps2)  "<VVMC_ACCComfortBandLower_mps2>"
  bus_selector4/29 -> outpmodule/386(VDDM_DCDCEnaDTC_raw32)  "<VDDM_DCDCEnaDTC_raw32>"
  bus_selector7/36 -> outpmodule/590(VDKC_UWB1Distance_enum)  "<VDKC_UWB1Distance_enum>"
  outpmodule/404(VOUTP_EDriveSysErrVCUErr_flg) -> bus_creator/404
  outpmodule/644(VOUTP_ReVehThdChkSta_enum) -> bus_creator/644
  bus_selector3/99 -> outpmodule/277(VBCM_AmbODAENFlash_enum)  "<VBCM_AmbODAENFlash_enum>"
  bus_selector10/11 -> outpmodule/631(VPMM_LVPwrSta_flg)  "<VPMM_LVPwrSta_flg>"
  bus_selector2/4 -> outpmodule/7(VAPM_FSOffSwTimeOut_flg)  "<VAPM_FSOffSwTimeOut_flg>"
  bus_selector12/131 -> outpmodule/842(VTHC_FDCTHCCREVentZStaSet3_enum)  "<VTHC_FDCTHCCREVentZStaSet3_enum>"
  bus_selector12/129 -> outpmodule/840(VTHC_FDCTHCCREVentZStaSet1_enum)  "<VTHC_FDCTHCCREVentZStaSet1_enum>"
  BAPM_outputs/1 -> bus_selector2/1
  bus_selector7/50 -> outpmodule/604(VDKC_JudgeKeepUnlockZone_flg)  "<VDKC_JudgeKeepUnlockZone_flg>"
  outpmodule/1066(VOUTP_VMCCCCtrlAvail_flg) -> bus_creator/1066
  bus_selector3/80 -> outpmodule/258(VBCM_PsRWdwCtrlCmd_pct)  "<VBCM_PsRWdwCtrlCmd_pct>"
  bus_selector12/127 -> outpmodule/838(VTHC_FDCTHCREVentZStaSet5_enum)  "<VTHC_FDCTHCREVentZStaSet5_enum>"
  bus_selector12/128 -> outpmodule/839(VTHC_FDCTHCREVentZStaSet7_enum)  "<VTHC_FDCTHCREVentZStaSet7_enum>"
  outpmodule/835(VOUTP_FDCTHCREVentZStaSet2_enum) -> bus_creator/835
  outpmodule/1166(VOUTP_CalibratedGyroX_Dps) -> bus_creator/1166
  bus_selector17/54 -> outpmodule/1113(VVMC_ADASFltWrnReq_flg)  "<VVMC_ADASFltWrnReq_flg>"
  bus_selector12/126 -> outpmodule/837(VTHC_FDCTHCREVentZStaSet4_enum)  "<VTHC_FDCTHCREVentZStaSet4_enum>"
  bus_selector4/127 -> outpmodule/484(VDDM_C1EPAS2LCDTC_raw32)  "<VDDM_C1EPAS2LCDTC_raw32>"
  bus_selector12/123 -> outpmodule/834(VTHC_FDCTHCREVentZStaSet1_enum)  "<VTHC_FDCTHCREVentZStaSet1_enum>"
  bus_selector17/61 -> outpmodule/1120(VVMC_ADASSLIFSpdLim_enum)  "<VVMC_ADASSLIFSpdLim_enum>"
  bus_selector7/33 -> outpmodule/587(VDKC_ReVehData_enum)  "<VDKC_ReVehData_enum>"
  bus_selector4/66 -> outpmodule/423(VDDM_FMRUSSDTC_raw32)  "<VDDM_FMRUSSDTC_raw32>"
  bus_selector12/121 -> outpmodule/832(VTHC_FDCTHCCLEVentZStaSet5_enum)  "<VTHC_FDCTHCCLEVentZStaSet5_enum>"
  bus_selector12/124 -> outpmodule/835(VTHC_FDCTHCREVentZStaSet2_enum)  "<VTHC_FDCTHCREVentZStaSet2_enum>"
  bus_selector17/45 -> outpmodule/1104(VVMC_ADASVehSpdLim_raw32)  "<VVMC_ADASVehSpdLim_raw32>"
  bus_selector12/125 -> outpmodule/836(VTHC_FDCTHCREVentZStaSet3_enum)  "<VTHC_FDCTHCREVentZStaSet3_enum>"
  outpmodule/4(VOUTP_VehSpeed_kph) -> bus_creator/4
  outpmodule/484(VOUTP_C1EPAS2LCDTC_raw32) -> bus_creator/484
  outpmodule/3(VOUTP_VehHVPwrAvail4THCM_W) -> bus_creator/3
  bus_selector12/47 -> outpmodule/758(VTHC_ACForceOFF_flg)  "<VTHC_ACForceOFF_flg>"
  outpmodule/2(VOUTP_LVBattVoltSta_enum) -> bus_creator/2
  outpmodule/751(VOUTP_ACModeMem_enum) -> bus_creator/751
  bus_selector3/38 -> outpmodule/216(VBCM_RrDefog_flg)  "<VBCM_RrDefog_flg>"
  outpmodule/142(VOUTP_AVMParkingmodeTimeOut_flg) -> bus_creator/142
  outpmodule/1(VOUTP_HVTHCMSysAvail_enum) -> bus_creator/1
  outpmodule/740(VOUTP_sigRecircSt_flg) -> bus_creator/740
  outpmodule/516(VOUTP_RegenErrDTC_raw32) -> bus_creator/516
  outpmodule/371(VOUTP_C1ABM1CSDTC_raw32) -> bus_creator/371
  outpmodule/311(VOUTP_WalkInUnLkENFunSta_flg) -> bus_creator/311
  outpmodule/853(VOUTP_FDCTHCCLEVentYStaSet2_enum) -> bus_creator/853
  outpmodule/1100(VOUTP_ACCJerkUpperLimit_mps3) -> bus_creator/1100
  outpmodule/373(VOUTP_Lv1ErrDTC_raw32) -> bus_creator/373
  bus_selector4/87 -> outpmodule/444(VDDM_BMSSigErrDetDTC_raw32)  "<VDDM_BMSSigErrDetDTC_raw32>"
  outpmodule/353(VOUTP_CLWinLockDrStaMem_enum) -> bus_creator/353
  bus_selector4/11 -> outpmodule/368(VDDM_C3CCU2CSDTC_raw32)  "<VDDM_C3CCU2CSDTC_raw32>"
  outpmodule/1065(VOUTP_VMCACCCtrlAvail_flg) -> bus_creator/1065
  outpmodule/350(VOUTP_DrRWdwReqAP_enum) -> bus_creator/350
  outpmodule/352(VOUTP_CLWinLockDrSta_flg) -> bus_creator/352
  bus_selector13/82 -> outpmodule/969(VTPM_Flashchkdatavalid_enum)  "<VTPM_Flashchkdatavalid_enum>"
  bus_selector4/19 -> outpmodule/376(VDDM_Lv4ErrDTC_raw32)  "<VDDM_Lv4ErrDTC_raw32>"
  bus_selector3/36 -> outpmodule/214(VBCM_MirrorCtrl_enum)  "<VBCM_MirrorCtrl_enum>"
  outpmodule/349(VOUTP_PasWdwReqAP_enum) -> bus_creator/349
  bus_selector3/132 -> outpmodule/310(VBCM_FollowMeENMem_enum)  "<VBCM_FollowMeENMem_enum>"
  BNMM_outputs/1 -> bus_selector9/1
  outpmodule/801(VOUTP_AirIntenZone1MSet5_enum) -> bus_creator/801
  outpmodule/346(VOUTP_HMIKey8FuncSta_enum) -> bus_creator/346
  outpmodule/347(VOUTP_AutoWipHSpdENSta_flg) -> bus_creator/347
  bus_selector3/67 -> outpmodule/245(VBCM_SPTGDet_flg)  "<VBCM_SPTGDet_flg>"
  outpmodule/345(VOUTP_HMIKey7FuncSta_enum) -> bus_creator/345
  bus_selector2/15 -> outpmodule/18(VAPM_APSDRLL_cm)  "<VAPM_APSDRLL_cm>"
  outpmodule/341(VOUTP_HMIKey3FuncSta_enum) -> bus_creator/341
  outpmodule/87(VOUTP_ShifterHandleCmd_enum) -> bus_creator/87
  outpmodule/880(VOUTP_FrostSet_enum) -> bus_creator/880
  outpmodule/342(VOUTP_HMIKey4FuncSta_enum) -> bus_creator/342
  bus_selector12/51 -> outpmodule/762(VTHC_sigSetTempZon2StM_C)  "<VTHC_sigSetTempZon2StM_C>"
  bus_selector3/56 -> outpmodule/234(VBCM_AmbLightBrightness3_enum)  "<VBCM_AmbLightBrightness3_enum>"
  bus_selector3/21 -> outpmodule/199(VBCM_DimmerEN_flg)  "<VBCM_DimmerEN_flg>"
  bus_selector4/151 -> outpmodule/508(VDDM_CAN2BusErrorDTC_raw32)  "<VDDM_CAN2BusErrorDTC_raw32>"
  outpmodule/727(VOUTP_FDFrLeAPTCHeatPwrCmd_W) -> bus_creator/727
  outpmodule/368(VOUTP_C3CCU2CSDTC_raw32) -> bus_creator/368
  bus_selector12/70 -> outpmodule/781(VTHC_FDCFGSChSta_enum)  "<VTHC_FDCFGSChSta_enum>"
  outpmodule/537(VOUTP_IPSAL_sec) -> bus_creator/537
  outpmodule/363(VOUTP_C3BMS1LCDTC_raw32) -> bus_creator/363
  outpmodule/951(VOUTP_ID4messageALTU_raw8) -> bus_creator/951
  outpmodule/261(VOUTP_AmbWelEN_flg) -> bus_creator/261
  outpmodule/262(VOUTP_AmbDimEN_flg) -> bus_creator/262
  bus_selector4/47 -> outpmodule/404(VDDM_EDriveSysErrVCUErr_flg)  "<VDDM_EDriveSysErrVCUErr_flg>"
  bus_selector2/158 -> outpmodule/161(VAPM_APSExitCondition_enum)  "<VAPM_APSExitCondition_enum>"
  outpmodule/260(VOUTP_AmbFunEN_flg) -> bus_creator/260
  outpmodule/307(VOUTP_WalkOutLkENMem_enum) -> bus_creator/307
  outpmodule/546(VOUTP_QTYPSATRIPSL_cnt) -> bus_creator/546
  outpmodule/354(VOUTP_WinLFOpenedSta_pct) -> bus_creator/354
  outpmodule/544(VOUTP_CDEODTL_km) -> bus_creator/544
  outpmodule/1150(VOUTP_APSCtrlAvail_flg) -> bus_creator/1150
  outpmodule/259(VOUTP_APMDoorControlSta_flg) -> bus_creator/259
  bus_selector3/73 -> outpmodule/251(VBCM_MirrorFlodPos_flg)  "<VBCM_MirrorFlodPos_flg>"
  outpmodule/251(VOUTP_MirrorFlodPos_flg) -> bus_creator/251
  bus_selector12/133 -> outpmodule/844(VTHC_FDCTHCCREVentZStaSet5_enum)  "<VTHC_FDCTHCCREVentZStaSet5_enum>"
  outpmodule/351(VOUTP_PsRWdwReqAP_enum) -> bus_creator/351
  outpmodule/257(VOUTP_DrRWdwCtrlCmd_pct) -> bus_creator/257
  bus_selector13/7 -> outpmodule/894(VTPM_LRWheelPress_raw8)  "<VTPM_LRWheelPress_raw8>"
  bus_selector12/115 -> outpmodule/826(VTHC_FDCTHCLEVentZStaSet5_enum)  "<VTHC_FDCTHCLEVentZStaSet5_enum>"
  outpmodule/583(VOUTP_UWBDetPTGArea_enum) -> bus_creator/583
  bus_selector2/152 -> outpmodule/155(VAPM_DriverSeatBeltCmd_flg)  "<VAPM_DriverSeatBeltCmd_flg>"
  outpmodule/258(VOUTP_PsRWdwCtrlCmd_pct) -> bus_creator/258
  outpmodule/782(VOUTP_FDCFGSAirIntCmd_enum) -> bus_creator/782
  bus_selector12/98 -> outpmodule/809(VTHC_IONSWStaSet_enum)  "<VTHC_IONSWStaSet_enum>"
  outpmodule/256(VOUTP_PasWdwCtrlCmd_pct) -> bus_creator/256
  outpmodule/104(VOUTP_GRADETimeOut_flg) -> bus_creator/104
  outpmodule/309(VOUTP_LockSettingStaMem_enum) -> bus_creator/309
  bus_selector14/51 -> outpmodule/1035(VTQD_SetSpd_kph)  "<VTQD_SetSpd_kph>"
  outpmodule/1036(VOUTP_VehActSpd_kph) -> bus_creator/1036
  outpmodule/1038(VOUTP_SetSpdLimWarn_flg) -> bus_creator/1038
  outpmodule/716(VOUTP_FDEXV1Cmd_step) -> bus_creator/716
  bus_selector17/64 -> outpmodule/1123(VVMC_ADASLFCSta_enum)  "<VVMC_ADASLFCSta_enum>"
  outpmodule/568(VOUTP_UWB4Invalid_flg) -> bus_creator/568
  outpmodule/615(VOUTP_PNI_flg) -> bus_creator/615
  outpmodule/1125(VOUTP_ADASLaneModeR_enum) -> bus_creator/1125
  outpmodule/254(VOUTP_PTGInnerSW2_enum) -> bus_creator/254
  outpmodule/946(VOUTP_S3WheelDebugALTU_pct) -> bus_creator/946
  bus_selector4/30 -> outpmodule/387(VDDM_HiLvSaChkDTC_raw32)  "<VDDM_HiLvSaChkDTC_raw32>"
  outpmodule/70(VOUTP_RRWhlRotDirTimeOut_flg) -> bus_creator/70
  outpmodule/268(VOUTP_LockAlarm_enum) -> bus_creator/268
  outpmodule/755(VOUTP_FaceM_flg) -> bus_creator/755
  outpmodule/692(VOUTP_SHA3_cnt) -> bus_creator/692
  bus_selector3/32 -> outpmodule/210(VBCM_HazardSW_flg)  "<VBCM_HazardSW_flg>"
  bus_selector2/84 -> outpmodule/87(VAPM_ShifterHandleCmd_enum)  "<VAPM_ShifterHandleCmd_enum>"
  outpmodule/1116(VOUTP_ACCTakeoverReq_flg) -> bus_creator/1116
  bus_selector2/83 -> outpmodule/86(VAPM_RRPulseCountTimeOut_flg)  "<VAPM_RRPulseCountTimeOut_flg>"
  outpmodule/1001(VOUTP_FrEDURolRgnTq_Nm) -> bus_creator/1001
  outpmodule/292(VOUTP_PassSWSta_flg) -> bus_creator/292
  bus_selector7/42 -> outpmodule/596(VDKC_UWB0FPP_enum)  "<VDKC_UWB0FPP_enum>"
  bus_selector3/179 -> outpmodule/357(VBCM_WinRROpenedSta_pct)  "<VBCM_WinRROpenedSta_pct>"
  bus_selector9/2 -> outpmodule/610(VNMM_NMmTxReq_flg)  "<VNMM_NMmTxReq_flg>"
  outpmodule/582(VOUTP_CalDistance_enum) -> bus_creator/582
  outpmodule/1110(VOUTP_LeftTurnLightReq_flg) -> bus_creator/1110
  bus_selector3/176 -> outpmodule/354(VBCM_WinLFOpenedSta_pct)  "<VBCM_WinLFOpenedSta_pct>"
  bus_selector3/178 -> outpmodule/356(VBCM_WinLROpenedSta_pct)  "<VBCM_WinLROpenedSta_pct>"
  outpmodule/1109(VOUTP_RightTurnLightReq_flg) -> bus_creator/1109
  outpmodule/982(VOUTP_TPMSSensorIDRegStart_flg) -> bus_creator/982
  bus_selector3/177 -> outpmodule/355(VBCM_WinRFOpenedSta_pct)  "<VBCM_WinRFOpenedSta_pct>"
  outpmodule/873(VOUTP_SettempZon1Set4_enum) -> bus_creator/873
  bus_selector3/173 -> outpmodule/351(VBCM_PsRWdwReqAP_enum)  "<VBCM_PsRWdwReqAP_enum>"
  outpmodule/88(VOUTP_ShifterHandleCmdTimeOut_flg) -> bus_creator/88
  bus_selector3/174 -> outpmodule/352(VBCM_CLWinLockDrSta_flg)  "<VBCM_CLWinLockDrSta_flg>"
  bus_selector3/166 -> outpmodule/344(VBCM_HMIKey6FuncSta_enum)  "<VBCM_HMIKey6FuncSta_enum>"
  outpmodule/1051(VOUTP_RrRateLimitInc_Nm) -> bus_creator/1051
  outpmodule/71(VOUTP_LFPulseCountV_flg) -> bus_creator/71
  bus_selector3/167 -> outpmodule/345(VBCM_HMIKey7FuncSta_enum)  "<VBCM_HMIKey7FuncSta_enum>"
  bus_selector3/164 -> outpmodule/342(VBCM_HMIKey4FuncSta_enum)  "<VBCM_HMIKey4FuncSta_enum>"
  outpmodule/757(VOUTP_CCUSyncSts_flg) -> bus_creator/757
  outpmodule/985(VOUTP_ParkRequest_flg) -> bus_creator/985
  outpmodule/673(VOUTP_CarModel2_cnt) -> bus_creator/673
  bus_selector7/20 -> outpmodule/574(VDKC_UIDBatVolt_enum)  "<VDKC_UIDBatVolt_enum>"
  bus_selector12/130 -> outpmodule/841(VTHC_FDCTHCCREVentZStaSet2_enum)  "<VTHC_FDCTHCCREVentZStaSet2_enum>"
  bus_selector11/9 -> outpmodule/677(VSYS_Major1_cnt)  "<VSYS_Major1_cnt>"
  bus_selector3/163 -> outpmodule/341(VBCM_HMIKey3FuncSta_enum)  "<VBCM_HMIKey3FuncSta_enum>"
  outpmodule/831(VOUTP_FDCTHCCLEVentZStaSet4_enum) -> bus_creator/831
  bus_selector3/162 -> outpmodule/340(VBCM_HMIKey2FuncSta_enum)  "<VBCM_HMIKey2FuncSta_enum>"
  bus_selector6/20 -> outpmodule/545(VDID_QTYPSATRIPSR_cnt)  "<VDID_QTYPSATRIPSR_cnt>"
  bus_selector12/88 -> outpmodule/799(VTHC_AirIntenZone1MSet3_enum)  "<VTHC_AirIntenZone1MSet3_enum>"
  outpmodule/893(VOUTP_RFWheelPress_raw8) -> bus_creator/893
  bus_selector3/160 -> outpmodule/338(VBCM_AutoUnlockMem_enum)  "<VBCM_AutoUnlockMem_enum>"
  outpmodule/280(VOUTP_AmbColorSta3_enum) -> bus_creator/280
  outpmodule/26(VOUTP_PASAFMR_enum) -> bus_creator/26
  bus_selector3/161 -> outpmodule/339(VBCM_HMIKey1FuncSta_enum)  "<VBCM_HMIKey1FuncSta_enum>"
  bus_selector2/95 -> outpmodule/98(VAPM_SASSpeedValidTimeOut_flg)  "<VAPM_SASSpeedValidTimeOut_flg>"
  outpmodule/786(VOUTP_FDCFGSIONCmd_flg) -> bus_creator/786
  bus_selector12/37 -> outpmodule/748(VTHC_sigCbnAirT_C)  "<VTHC_sigCbnAirT_C>"
  outpmodule/863(VOUTP_FDCTHCREVentYStaSet7_enum) -> bus_creator/863
  outpmodule/1106(VOUTP_ADASShftPosnReq_enum) -> bus_creator/1106
  bus_selector4/35 -> outpmodule/392(VDDM_MCUActDTC_raw32)  "<VDDM_MCUActDTC_raw32>"
  bus_selector13/91 -> outpmodule/978(VTPM_FlashIDvalid_enum)  "<VTPM_FlashIDvalid_enum>"
  bus_selector3/158 -> outpmodule/336(VBCM_AutoLockMem_enum)  "<VBCM_AutoLockMem_enum>"
  bus_selector3/157 -> outpmodule/335(VBCM_AutoLockSta_flg)  "<VBCM_AutoLockSta_flg>"
  outpmodule/507(VOUTP_CAN1BusErrorDTC_raw32) -> bus_creator/507
  bus_selector3/156 -> outpmodule/334(VBCM_LLeftStaCmd_flg)  "<VBCM_LLeftStaCmd_flg>"
  bus_selector3/155 -> outpmodule/333(VBCM_LRightStaCmd_flg)  "<VBCM_LRightStaCmd_flg>"
  bus_selector3/154 -> outpmodule/332(VBCM_ACCLevelMem57_enum)  "<VBCM_ACCLevelMem57_enum>"
  bus_selector10/30 -> outpmodule/650(VPMM_SilentChkAllowSleep_flg)  "<VPMM_SilentChkAllowSleep_flg>"
  bus_selector4/15 -> outpmodule/372(VDDM_C1ABM1LCDTC_raw32)  "<VDDM_C1ABM1LCDTC_raw32>"
  bus_selector3/150 -> outpmodule/328(VBCM_SenstivityPosnCmd_enum)  "<VBCM_SenstivityPosnCmd_enum>"
  outpmodule/699(VOUTP_FdcSlpReqRisingEdge_flg) -> bus_creator/699
  bus_selector7/34 -> outpmodule/588(VDKC_UWB0Distance_enum)  "<VDKC_UWB0Distance_enum>"
  bus_selector7/41 -> outpmodule/595(VDKC_BLEdcEvent_enum)  "<VDKC_BLEdcEvent_enum>"
  outpmodule/563(VOUTP_DkeyShowIVISta_enum) -> bus_creator/563
  bus_selector10/3 -> outpmodule/623(VPMM_PowerUpFault_enum)  "<VPMM_PowerUpFault_enum>"
  bus_selector3/152 -> outpmodule/330(VBCM_ACCLevelMem12_enum)  "<VBCM_ACCLevelMem12_enum>"
  bus_selector3/151 -> outpmodule/329(VBCM_TimeGapLevelSta_enum)  "<VBCM_TimeGapLevelSta_enum>"
  outpmodule/136(VOUTP_EPBStaTimeOut_flg) -> bus_creator/136
  bus_selector10/33 -> outpmodule/653(VPMM_PMMAllowECUSleep_flg)  "<VPMM_PMMAllowECUSleep_flg>"
  outpmodule/955(VOUTP_ChkStorge_flg) -> bus_creator/955
  bus_selector12/19 -> outpmodule/730(VTHC_FDBlowerCmd_pct)  "<VTHC_FDBlowerCmd_pct>"
  bus_selector12/165 -> outpmodule/876(VTHC_ACModeSet123_enum)  "<VTHC_ACModeSet123_enum>"
  outpmodule/510(VOUTP_CAN4BusErrorDTC_raw32) -> bus_creator/510
  bus_selector3/148 -> outpmodule/326(VBCM_PTGOpenHeight34_enum)  "<VBCM_PTGOpenHeight34_enum>"
  outpmodule/797(VOUTP_AirIntenZone1MSet1_enum) -> bus_creator/797
  bus_selector12/56 -> outpmodule/767(VTHC_FDCTHCLEVentZSta_enum)  "<VTHC_FDCTHCLEVentZSta_enum>"
  outpmodule/195(VOUTP_CTDCtrl_enum) -> bus_creator/195
  outpmodule/783(VOUTP_FDCFGSFuncSta_enum) -> bus_creator/783
  bus_selector12/35 -> outpmodule/746(VTHC_sigCbnSolarRight_W)  "<VTHC_sigCbnSolarRight_W>"
  outpmodule/1032(VOUTP_FDCVCURegenMode_enum) -> bus_creator/1032
  outpmodule/472(VOUTP_LFPressIndiDTC_raw32) -> bus_creator/472
  bus_selector12/26 -> outpmodule/737(VTHC_CCUSyncLampSts_flg)  "<VTHC_CCUSyncLampSts_flg>"
  bus_selector5/2 -> outpmodule/518(VDHP_LowIdleAccPedal_flg)  "<VDHP_LowIdleAccPedal_flg>"
  bus_selector13/5 -> outpmodule/892(VTPM_LFWheelPress_raw8)  "<VTPM_LFWheelPress_raw8>"
  outpmodule/1126(VOUTP_ADASSLIFSta_enum) -> bus_creator/1126
  bus_selector17/30 -> outpmodule/1089(VVMC_LKATOIFault_flg)  "<VVMC_LKATOIFault_flg>"
  bus_selector3/72 -> outpmodule/250(VBCM_MFSWTri_flg)  "<VBCM_MFSWTri_flg>"
  outpmodule/377(VOUTP_BrkSWErrDTC_raw32) -> bus_creator/377
  outpmodule/1030(VOUTP_OPDHoldLamp_flg) -> bus_creator/1030
  outpmodule/1031(VOUTP_SaveRegenMode_enum) -> bus_creator/1031
  bus_selector3/171 -> outpmodule/349(VBCM_PasWdwReqAP_enum)  "<VBCM_PasWdwReqAP_enum>"
  outpmodule/571(VOUTP_UWB1Invalid_flg) -> bus_creator/571
  outpmodule/348(VOUTP_DrvWdwReqAP_enum) -> bus_creator/348
  outpmodule/1028(VOUTP_RegenTqLimitEn_flg) -> bus_creator/1028
  bus_selector4/73 -> outpmodule/430(VDDM_FLRUSSDTC_raw32)  "<VDDM_FLRUSSDTC_raw32>"
  bus_selector7/49 -> outpmodule/603(VDKC_FDCDKCAllowSleep_flg)  "<VDKC_FDCDKCAllowSleep_flg>"
  outpmodule/1029(VOUTP_IVIPwrLockSta_enum) -> bus_creator/1029
  outpmodule/958(VOUTP_RFPind_enum) -> bus_creator/958
  outpmodule/1026(VOUTP_DriveProtEn_flg) -> bus_creator/1026
  outpmodule/771(VOUTP_FDCTHCLEVentYSta_enum) -> bus_creator/771
  outpmodule/1033(VOUTP_SpdCtrlMode_enum) -> bus_creator/1033
  bus_selector17/33 -> outpmodule/1092(VVMC_ADASFaultSta_flg)  "<VVMC_ADASFaultSta_flg>"
  outpmodule/813(VOUTP_FDCFGSAirIntStaSet457_enum) -> bus_creator/813
  outpmodule/255(VOUTP_DrvWdwCtrlCmd_pct) -> bus_creator/255
  outpmodule/310(VOUTP_FollowMeENMem_enum) -> bus_creator/310
  outpmodule/464(VOUTP_ESC5RCErrDTC_raw32) -> bus_creator/464
  bus_selector3/53 -> outpmodule/231(VBCM_AmbLightBreath6_enum)  "<VBCM_AmbLightBreath6_enum>"
  outpmodule/1024(VOUTP_RDCActive_enum) -> bus_creator/1024
  outpmodule/212(VOUTP_RTurnLP_flg) -> bus_creator/212
  bus_selector7/46 -> outpmodule/600(VDKC_UWB4FPP_enum)  "<VDKC_UWB4FPP_enum>"
  outpmodule/1104(VOUTP_ADASVehSpdLim_raw32) -> bus_creator/1104
  bus_selector13/53 -> outpmodule/940(VTPM_LRP20_raw8)  "<VTPM_LRP20_raw8>"
  outpmodule/357(VOUTP_WinRROpenedSta_pct) -> bus_creator/357
  bus_selector3/134 -> outpmodule/312(VBCM_WalkOutLkENFunSta_flg)  "<VBCM_WalkOutLkENFunSta_flg>"
  outpmodule/1023(VOUTP_CreepON_flg) -> bus_creator/1023
  bus_selector2/39 -> outpmodule/42(VAPM_SNSRLayout_enum)  "<VAPM_SNSRLayout_enum>"
  outpmodule/1025(VOUTP_EquivAccPedalSWSta_flg) -> bus_creator/1025
  bus_selector3/7 -> outpmodule/185(VBCM_HoodSW_flg)  "<VBCM_HoodSW_flg>"
  outpmodule/726(VOUTP_FDEWP3Cmd_enum) -> bus_creator/726
  bus_selector12/49 -> outpmodule/760(VTHC_AirIntenZone1M_enum)  "<VTHC_AirIntenZone1M_enum>"
  outpmodule/1130(VOUTP_ADASLFCHandsOffWarning_enum) -> bus_creator/1130
  outpmodule/1020(VOUTP_RrUdcMax_V) -> bus_creator/1020
  outpmodule/401(VOUTP_RRDoorSWDTC_raw32) -> bus_creator/401
  outpmodule/1021(VOUTP_ReBrakeLPReq_flg) -> bus_creator/1021
  outpmodule/885(VOUTP_FDCFGSLearnCmd_enum) -> bus_creator/885
  bus_selector2/108 -> outpmodule/111(VAPM_MCPressure_bar)  "<VAPM_MCPressure_bar>"
  outpmodule/1022(VOUTP_BOSEnable_flg) -> bus_creator/1022
  bus_selector2/86 -> outpmodule/89(VAPM_DriIntend_enum)  "<VAPM_DriIntend_enum>"
  bus_selector3/17 -> outpmodule/195(VBCM_CTDCtrl_enum)  "<VBCM_CTDCtrl_enum>"
  outpmodule/1019(VOUTP_RrUdcMin_V) -> bus_creator/1019
  bus_selector13/70 -> outpmodule/957(VTPM_LFPindi_enum)  "<VTPM_LFPindi_enum>"
  bus_selector4/8 -> outpmodule/365(VDDM_C3CCU1CSDTC_raw32)  "<VDDM_C3CCU1CSDTC_raw32>"
  outpmodule/288(VOUTP_AmbBrightnessSta5_enum) -> bus_creator/288
  outpmodule/188(VOUTP_PsDoorSW_flg) -> bus_creator/188
  outpmodule/1017(VOUTP_RrIdcMin_A) -> bus_creator/1017
  outpmodule/1111(VOUTP_ADASFCWSta_enum) -> bus_creator/1111
  outpmodule/1015(VOUTP_FrUdcMin_V) -> bus_creator/1015
  bus_selector2/154 -> outpmodule/157(VAPM_APSProgressPCT_pct)  "<VAPM_APSProgressPCT_pct>"
  outpmodule/724(VOUTP_FDEWP1Cmd_enum) -> bus_creator/724
  bus_selector2/36 -> outpmodule/39(VAPM_USSStaFCR_flg)  "<VAPM_USSStaFCR_flg>"
  outpmodule/344(VOUTP_HMIKey6FuncSta_enum) -> bus_creator/344
  outpmodule/1016(VOUTP_FrUdcMax_V) -> bus_creator/1016
  bus_selector12/102 -> outpmodule/813(VTHC_FDCFGSAirIntStaSet457_enum)  "<VTHC_FDCFGSAirIntStaSet457_enum>"
  outpmodule/364(VOUTP_C3CCU1RCDTC_raw32) -> bus_creator/364
  outpmodule/1014(VOUTP_FrIdcMax_A) -> bus_creator/1014
  bus_selector12/90 -> outpmodule/801(VTHC_AirIntenZone1MSet5_enum)  "<VTHC_AirIntenZone1MSet5_enum>"
  bus_selector2/96 -> outpmodule/99(VAPM_SASCAL_flg)  "<VAPM_SASCAL_flg>"
  outpmodule/1013(VOUTP_FrIdcMin_A) -> bus_creator/1013
  outpmodule/1012(VOUTP_RrRgnPermSta_flg) -> bus_creator/1012
  bus_selector12/100 -> outpmodule/811(VTHC_FDCFGSChStaSet457_enum)  "<VTHC_FDCFGSChStaSet457_enum>"
  bus_selector4/137 -> outpmodule/494(VDDM_VCURAPSErrLv3_flg)  "<VDDM_VCURAPSErrLv3_flg>"
  bus_selector2/47 -> outpmodule/50(VAPM_RFRawWhlSpeedTimeOut_flg)  "<VAPM_RFRawWhlSpeedTimeOut_flg>"
  outpmodule/372(VOUTP_C1ABM1LCDTC_raw32) -> bus_creator/372
  outpmodule/1011(VOUTP_FrRgnPermSta_flg) -> bus_creator/1011
  bus_selector3/143 -> outpmodule/321(VBCM_PTGUserHeight3_cnt)  "<VBCM_PTGUserHeight3_cnt>"
  bus_selector3/79 -> outpmodule/257(VBCM_DrRWdwCtrlCmd_pct)  "<VBCM_DrRWdwCtrlCmd_pct>"
  bus_selector17/115 -> outpmodule/1174(VVMC_FDCVMCMaxAngCtrlOutTqLim_Nm)  "<VVMC_FDCVMCMaxAngCtrlOutTqLim_Nm>"
  bus_selector13/56 -> outpmodule/943(VTPM_IDin_raw32)  "<VTPM_IDin_raw32>"
  outpmodule/1010(VOUTP_PTCSPermSta_flg) -> bus_creator/1010
  outpmodule/654(VOUTP_LVSilentChrgSta_enum) -> bus_creator/654
  outpmodule/1009(VOUTP_RgnAbnorSta_flg) -> bus_creator/1009
  outpmodule/1008(VOUTP_RrEDUAvailBrkRgnTqV_flg) -> bus_creator/1008
  outpmodule/265(VOUTP_AmbODAEN_flg) -> bus_creator/265
  outpmodule/688(VOUTP_Change2_cnt) -> bus_creator/688
  outpmodule/283(VOUTP_AmbColorSta7_enum) -> bus_creator/283
  outpmodule/876(VOUTP_ACModeSet123_enum) -> bus_creator/876
  bus_selector4/115 -> outpmodule/472(VDDM_LFPressIndiDTC_raw32)  "<VDDM_LFPressIndiDTC_raw32>"
  outpmodule/974(VOUTP_FlashS1ID_raw) -> bus_creator/974
  bus_selector17/56 -> outpmodule/1115(VVMC_ForceLowBeam_enum)  "<VVMC_ForceLowBeam_enum>"
  outpmodule/1089(VOUTP_LKATOIFault_flg) -> bus_creator/1089
  outpmodule/1007(VOUTP_RrEDUSpdValid_flg) -> bus_creator/1007
  outpmodule/790(VOUTP_EWPBUflag3_flg) -> bus_creator/790
  outpmodule/1006(VOUTP_FrEDUAvailBrkRgnTqV_flg) -> bus_creator/1006
  outpmodule/293(VOUTP_FWipSwSta_enum) -> bus_creator/293
  outpmodule/696(VOUTP_SHA7_cnt) -> bus_creator/696
  outpmodule/903(VOUTP_RRSensorFail_flg) -> bus_creator/903
  outpmodule/1050(VOUTP_FrRateLimitDec_Nm) -> bus_creator/1050
  outpmodule/1004(VOUTP_RrEDUSpd_rpm) -> bus_creator/1004
  outpmodule/1087(VOUTP_ADASLKASta_enum) -> bus_creator/1087
  outpmodule/1005(VOUTP_FrEDUSpdValid_flg) -> bus_creator/1005
  outpmodule/275(VOUTP_AmbLinkDriStaFlash_enum) -> bus_creator/275
  bus_selector14/45 -> outpmodule/1029(VTQD_IVIPwrLockSta_enum)  "<VTQD_IVIPwrLockSta_enum>"
  outpmodule/857(VOUTP_FDCTHCCLEVentYStaSet7_enum) -> bus_creator/857
  bus_selector13/14 -> outpmodule/901(VTPM_RFSensorFail_flg)  "<VTPM_RFSensorFail_flg>"
  bus_selector14/32 -> outpmodule/1016(VTQD_FrUdcMax_V)  "<VTQD_FrUdcMax_V>"
  bus_selector7/25 -> outpmodule/579(VDKC_CoordinateY_enum)  "<VDKC_CoordinateY_enum>"
  bus_selector2/167 -> outpmodule/170(VAPM_APSShiftPosnReq_enum)  "<VAPM_APSShiftPosnReq_enum>"
  bus_selector14/29 -> outpmodule/1013(VTQD_FrIdcMin_A)  "<VTQD_FrIdcMin_A>"
  bus_selector17/14 -> outpmodule/1073(VVMC_RearWhlSlipRatioCtrl_flg)  "<VVMC_RearWhlSlipRatioCtrl_flg>"
  bus_selector14/30 -> outpmodule/1014(VTQD_FrIdcMax_A)  "<VTQD_FrIdcMax_A>"
  outpmodule/303(VOUTP_FDRHandleLampCmd_flg) -> bus_creator/303
  bus_selector4/2 -> outpmodule/359(VDDM_C3BMS6CSDTC_raw32)  "<VDDM_C3BMS6CSDTC_raw32>"
  bus_selector2/14 -> outpmodule/17(VAPM_APSDRLR_cm)  "<VAPM_APSDRLR_cm>"
  bus_selector12/152 -> outpmodule/863(VTHC_FDCTHCREVentYStaSet7_enum)  "<VTHC_FDCTHCREVentYStaSet7_enum>"
  bus_selector14/28 -> outpmodule/1012(VTQD_RrRgnPermSta_flg)  "<VTQD_RrRgnPermSta_flg>"
  outpmodule/953(VOUTP_SetIDLoc_flg) -> bus_creator/953
  outpmodule/787(VOUTP_FDCTHCMPreWPTCHeatSta_enum) -> bus_creator/787
  bus_selector12/134 -> outpmodule/845(VTHC_FDCTHCCREVentZStaSet7_enum)  "<VTHC_FDCTHCCREVentZStaSet7_enum>"
  BTQD_outputs/1 -> bus_selector14/1
  bus_selector6/9 -> outpmodule/534(VDID_PSAR_sec)  "<VDID_PSAR_sec>"
  bus_selector14/26 -> outpmodule/1010(VTQD_PTCSPermSta_flg)  "<VTQD_PTCSPermSta_flg>"
  bus_selector12/5 -> outpmodule/716(VTHC_FDEXV1Cmd_step)  "<VTHC_FDEXV1Cmd_step>"
  bus_selector3/169 -> outpmodule/347(VBCM_AutoWipHSpdENSta_flg)  "<VBCM_AutoWipHSpdENSta_flg>"
  outpmodule/31(VOUTP_USSStaRLR_flg) -> bus_creator/31
  bus_selector4/3 -> outpmodule/360(VDDM_C3BMS6LCDTC_raw32)  "<VDDM_C3BMS6LCDTC_raw32>"
  outpmodule/730(VOUTP_FDBlowerCmd_pct) -> bus_creator/730
  bus_selector14/21 -> outpmodule/1005(VTQD_FrEDUSpdValid_flg)  "<VTQD_FrEDUSpdValid_flg>"
  outpmodule/607(VOUTP_DISCSta_enum) -> bus_creator/607
  bus_selector3/142 -> outpmodule/320(VBCM_PTGUserHeight2_cnt)  "<VBCM_PTGUserHeight2_cnt>"
  bus_selector7/37 -> outpmodule/591(VDKC_UWB2Distance_enum)  "<VDKC_UWB2Distance_enum>"
  outpmodule/567(VOUTP_KeyAreaPTG_enum) -> bus_creator/567
  outpmodule/1113(VOUTP_ADASFltWrnReq_flg) -> bus_creator/1113
  bus_selector14/24 -> outpmodule/1008(VTQD_RrEDUAvailBrkRgnTqV_flg)  "<VTQD_RrEDUAvailBrkRgnTqV_flg>"
  outpmodule/859(VOUTP_FDCTHCREVentYStaSet2_enum) -> bus_creator/859
  outpmodule/1057(VOUTP_ReqOBCIntrV2LEna_enum) -> bus_creator/1057
  outpmodule/9(VOUTP_PASDRMR_cm) -> bus_creator/9
  bus_selector14/23 -> outpmodule/1007(VTQD_RrEDUSpdValid_flg)  "<VTQD_RrEDUSpdValid_flg>"
  outpmodule/871(VOUTP_SettempZon1Set2_enum) -> bus_creator/871
  bus_selector12/24 -> outpmodule/735(VTHC_CCUAutoLampSts_flg)  "<VTHC_CCUAutoLampSts_flg>"
  bus_selector12/99 -> outpmodule/810(VTHC_FDCFGSChStaSet123_enum)  "<VTHC_FDCFGSChStaSet123_enum>"
  outpmodule/192(VOUTP_FrChargingDoorCtrl_enum) -> bus_creator/192
  bus_selector4/133 -> outpmodule/490(VDDM_DTCDetect_enum)  "<VDDM_DTCDetect_enum>"
  bus_selector14/20 -> outpmodule/1004(VTQD_RrEDUSpd_rpm)  "<VTQD_RrEDUSpd_rpm>"
  outpmodule/32(VOUTP_USSStaRLL_flg) -> bus_creator/32
  bus_selector14/22 -> outpmodule/1006(VTQD_FrEDUAvailBrkRgnTqV_flg)  "<VTQD_FrEDUAvailBrkRgnTqV_flg>"
  bus_selector3/16 -> outpmodule/194(VBCM_CrashDetd_flg)  "<VBCM_CrashDetd_flg>"
  outpmodule/86(VOUTP_RRPulseCountTimeOut_flg) -> bus_creator/86
  bus_selector12/156 -> outpmodule/867(VTHC_FDCTHCCREVentYStaSet4_enum)  "<VTHC_FDCTHCCREVentYStaSet4_enum>"
  outpmodule/674(VOUTP_CarModel3_cnt) -> bus_creator/674
  bus_selector14/19 -> outpmodule/1003(VTQD_FrEDUSpd_rpm)  "<VTQD_FrEDUSpd_rpm>"
  outpmodule/1027(VOUTP_ActParkRequest_flg) -> bus_creator/1027
  bus_selector2/139 -> outpmodule/142(VAPM_AVMParkingmodeTimeOut_flg)  "<VAPM_AVMParkingmodeTimeOut_flg>"
  outpmodule/552(VOUTP_VinCode_cnt) -> bus_creator/552
  bus_selector14/14 -> outpmodule/998(VTQD_DriverWhlTqDemRr_Nm)  "<VTQD_DriverWhlTqDemRr_Nm>"
  outpmodule/1128(VOUTP_ADASLDWMute_flg) -> bus_creator/1128
  bus_selector14/15 -> outpmodule/999(VTQD_FrEDUActTq_Nm)  "<VTQD_FrEDUActTq_Nm>"
  bus_selector2/98 -> outpmodule/101(VAPM_SASV_flg)  "<VAPM_SASV_flg>"
  bus_selector7/30 -> outpmodule/584(VDKC_A0UWBEvent_enum)  "<VDKC_A0UWBEvent_enum>"
  bus_selector12/122 -> outpmodule/833(VTHC_FDCTHCCLEVentZStaSet7_enum)  "<VTHC_FDCTHCCLEVentZStaSet7_enum>"
  bus_selector3/42 -> outpmodule/220(VBCM_TailgateHDSW_flg)  "<VBCM_TailgateHDSW_flg>"
  bus_selector14/18 -> outpmodule/1002(VTQD_RrEDURolRgnTq_Nm)  "<VTQD_RrEDURolRgnTq_Nm>"
  outpmodule/856(VOUTP_FDCTHCCLEVentYStaSet5_enum) -> bus_creator/856
  outpmodule/383(VOUTP_DCDC4PreDTC_raw32) -> bus_creator/383
  bus_selector14/17 -> outpmodule/1001(VTQD_FrEDURolRgnTq_Nm)  "<VTQD_FrEDURolRgnTq_Nm>"
  outpmodule/869(VOUTP_FDCTHCCREVentYStaSet7_enum) -> bus_creator/869
  bus_selector3/149 -> outpmodule/327(VBCM_PTGOpenHeight57_enum)  "<VBCM_PTGOpenHeight57_enum>"
  bus_selector14/16 -> outpmodule/1000(VTQD_RrEDUActTq_Nm)  "<VTQD_RrEDUActTq_Nm>"
  outpmodule/602(VOUTP_OutputPCMDModule_enum) -> bus_creator/602
  bus_selector4/153 -> outpmodule/510(VDDM_CAN4BusErrorDTC_raw32)  "<VDDM_CAN4BusErrorDTC_raw32>"
  bus_selector14/13 -> outpmodule/997(VTQD_DriverWhlTqDemFr_Nm)  "<VTQD_DriverWhlTqDemFr_Nm>"
  bus_selector8/3 -> outpmodule/607(VDSC_DISCSta_enum)  "<VDSC_DISCSta_enum>"
  bus_selector3/33 -> outpmodule/211(VBCM_LTurnLP_flg)  "<VBCM_LTurnLP_flg>"
  bus_selector14/12 -> outpmodule/996(VTQD_RrRgnDecrSta_flg)  "<VTQD_RrRgnDecrSta_flg>"
  bus_selector3/170 -> outpmodule/348(VBCM_DrvWdwReqAP_enum)  "<VBCM_DrvWdwReqAP_enum>"
  bus_selector14/10 -> outpmodule/994(VTQD_RrActvDmpDisabReq_flg)  "<VTQD_RrActvDmpDisabReq_flg>"
  outpmodule/379(VOUTP_KeyAuthDTC_raw32) -> bus_creator/379
  outpmodule/1174(VOUTP_FDCVMCMaxAngCtrlOutTqLim_Nm) -> bus_creator/1174
  bus_selector14/6 -> outpmodule/990(VTQD_EVDriveMode_enum)  "<VTQD_EVDriveMode_enum>"
  bus_selector12/58 -> outpmodule/769(VTHC_FDCTHCREVentZSta_enum)  "<VTHC_FDCTHCREVentZSta_enum>"
  bus_selector12/40 -> outpmodule/751(VTHC_ACModeMem_enum)  "<VTHC_ACModeMem_enum>"
  outpmodule/38(VOUTP_USSStaFLL_flg) -> bus_creator/38
  bus_selector12/142 -> outpmodule/853(VTHC_FDCTHCCLEVentYStaSet2_enum)  "<VTHC_FDCTHCCLEVentYStaSet2_enum>"
  outpmodule/576(VOUTP_FDCSPTGDet_flg) -> bus_creator/576
  outpmodule/1133(VOUTP_LVDAFailinfo_flg) -> bus_creator/1133
  bus_selector7/32 -> outpmodule/586(VDKC_KeyModeSta_enum)  "<VDKC_KeyModeSta_enum>"
  bus_selector14/5 -> outpmodule/989(VTQD_RrEDUAvailBrkRgnTq_Nm)  "<VTQD_RrEDUAvailBrkRgnTq_Nm>"
  bus_selector14/1 -> outpmodule/985(VTQD_ParkRequest_flg)  "<VTQD_ParkRequest_flg>"
  outpmodule/534(VOUTP_PSAR_sec) -> bus_creator/534
  outpmodule/547(VOUTP_PROTOCOLID_enum) -> bus_creator/547
  bus_selector17/59 -> outpmodule/1118(VVMC_ADASCAMSpdLim_enum)  "<VVMC_ADASCAMSpdLim_enum>"
  bus_selector11/43 -> outpmodule/711(VSYS_Var5_cnt)  "<VSYS_Var5_cnt>"
  outpmodule/549(VOUTP_ECUNAME_cnt) -> bus_creator/549
  bus_selector11/39 -> outpmodule/707(VSYS_PmicBootPath_raw32)  "<VSYS_PmicBootPath_raw32>"
  outpmodule/253(VOUTP_MFRDNBrightReq_pct) -> bus_creator/253
  bus_selector3/159 -> outpmodule/337(VBCM_AutoUnlockSta_flg)  "<VBCM_AutoUnlockSta_flg>"
  bus_selector11/40 -> outpmodule/708(VSYS_DrivingMode_cnt)  "<VSYS_DrivingMode_cnt>"
  outpmodule/13(VOUTP_PASDFMR_cm) -> bus_creator/13
  bus_selector11/41 -> outpmodule/709(VSYS_ModelYear_cnt)  "<VSYS_ModelYear_cnt>"
  bus_selector12/23 -> outpmodule/734(VTHC_CCUACLampSts_flg)  "<VTHC_CCUACLampSts_flg>"
  outpmodule/1153(VOUTP_APSDecReqA_flg) -> bus_creator/1153
  bus_selector3/165 -> outpmodule/343(VBCM_HMIKey5FuncSta_enum)  "<VBCM_HMIKey5FuncSta_enum>"
  bus_selector11/38 -> outpmodule/706(VSYS_ECUGen2_cnt)  "<VSYS_ECUGen2_cnt>"
  bus_selector13/43 -> outpmodule/930(VTPM_S2ID_raw32)  "<VTPM_S2ID_raw32>"
  outpmodule/220(VOUTP_TailgateHDSW_flg) -> bus_creator/220
  bus_selector11/35 -> outpmodule/703(VSYS_AcoreRebootCmdACK_flg)  "<VSYS_AcoreRebootCmdACK_flg>"
  bus_selector2/153 -> outpmodule/156(VAPM_DriverSeatBeltCmdTimeOut_flg)  "<VAPM_DriverSeatBeltCmdTimeOut_flg>"
  bus_selector11/30 -> outpmodule/698(VSYS_NvWriteReqRisingEdge_flg)  "<VSYS_NvWriteReqRisingEdge_flg>"
  bus_selector2/117 -> outpmodule/120(VAPM_MCPressureVTimeOut_flg)  "<VAPM_MCPressureVTimeOut_flg>"
  bus_selector4/111 -> outpmodule/468(VDDM_LFBatwarnDTC_raw32)  "<VDDM_LFBatwarnDTC_raw32>"
  bus_selector5/1 -> outpmodule/517(VDHP_ActAPSPosn_pct)  "<VDHP_ActAPSPosn_pct>"
  bus_selector11/29 -> outpmodule/697(VSYS_SHA8_cnt)  "<VSYS_SHA8_cnt>"
  outpmodule/991(VOUTP_ShiftGearPosn_enum) -> bus_creator/991
  outpmodule/1043(VOUTP_SimSoundCmd_pct) -> bus_creator/1043
  bus_selector2/11 -> outpmodule/14(VAPM_PASDFML_cm)  "<VAPM_PASDFML_cm>"
  bus_selector7/19 -> outpmodule/573(VDKC_UWB0Invalid_flg)  "<VDKC_UWB0Invalid_flg>"
  bus_selector2/147 -> outpmodule/150(VAPM_IVIScreenTimeOut_flg)  "<VAPM_IVIScreenTimeOut_flg>"
  outpmodule/138(VOUTP_AVMparkingcancelTimeOut_flg) -> bus_creator/138
  bus_selector11/28 -> outpmodule/696(VSYS_SHA7_cnt)  "<VSYS_SHA7_cnt>"
  bus_selector13/12 -> outpmodule/899(VTPM_RRWheelTemp_C)  "<VTPM_RRWheelTemp_C>"
  bus_selector3/153 -> outpmodule/331(VBCM_ACCLevelMem34_enum)  "<VBCM_ACCLevelMem34_enum>"
  bus_selector3/23 -> outpmodule/201(VBCM_LBeam_flg)  "<VBCM_LBeam_flg>"
  outpmodule/37(VOUTP_USSStaFLR_flg) -> bus_creator/37
  outpmodule/733(VOUTP_CabinMode_enum) -> bus_creator/733
  bus_selector11/26 -> outpmodule/694(VSYS_SHA5_cnt)  "<VSYS_SHA5_cnt>"
  outpmodule/1040(VOUTP_TrailerDisOPDSta_flg) -> bus_creator/1040
  bus_selector17/25 -> outpmodule/1084(VVMC_FeatArbitrFinal_enum)  "<VVMC_FeatArbitrFinal_enum>"
  bus_selector12/172 -> outpmodule/883(VTHC_RVentEN_flg)  "<VTHC_RVentEN_flg>"
  bus_selector3/62 -> outpmodule/240(VBCM_AmbLightColor3_enum)  "<VBCM_AmbLightColor3_enum>"
  bus_selector11/23 -> outpmodule/691(VSYS_SHA2_cnt)  "<VSYS_SHA2_cnt>"
  bus_selector3/147 -> outpmodule/325(VBCM_PTGOpenHeight12_enum)  "<VBCM_PTGOpenHeight12_enum>"
  bus_selector4/21 -> outpmodule/378(VDDM_BrkSWNoBacDTC_raw32)  "<VDDM_BrkSWNoBacDTC_raw32>"
  BSYS_outputs/1 -> bus_selector11/1
  bus_selector11/21 -> outpmodule/689(VSYS_Dash2_cnt)  "<VSYS_Dash2_cnt>"
  outpmodule/80(VOUTP_LFPulseCountTimeOut_flg) -> bus_creator/80
  outpmodule/247(VOUTP_FollowMe_flg) -> bus_creator/247
  bus_selector3/63 -> outpmodule/241(VBCM_AmbLightColor4_enum)  "<VBCM_AmbLightColor4_enum>"
  bus_selector11/42 -> outpmodule/710(VSYS_Var4_cnt)  "<VSYS_Var4_cnt>"
  bus_selector14/11 -> outpmodule/995(VTQD_FrRgnDecrSta_flg)  "<VTQD_FrRgnDecrSta_flg>"
  bus_selector14/31 -> outpmodule/1015(VTQD_FrUdcMin_V)  "<VTQD_FrUdcMin_V>"
  bus_selector11/20 -> outpmodule/688(VSYS_Change2_cnt)  "<VSYS_Change2_cnt>"
  bus_selector11/19 -> outpmodule/687(VSYS_Change1_cnt)  "<VSYS_Change1_cnt>"
  bus_selector11/22 -> outpmodule/690(VSYS_SHA1_cnt)  "<VSYS_SHA1_cnt>"
  bus_selector13/33 -> outpmodule/920(VTPM_LRWheelPSW_raw8)  "<VTPM_LRWheelPSW_raw8>"
  bus_selector12/66 -> outpmodule/777(VTHC_FDCTHCCREVentYSta_enum)  "<VTHC_FDCTHCCREVentYSta_enum>"
  bus_selector11/18 -> outpmodule/686(VSYS_Dash1_cnt)  "<VSYS_Dash1_cnt>"
  outpmodule/463(VOUTP_ESC1CSErrDTC_raw32) -> bus_creator/463
  outpmodule/860(VOUTP_FDCTHCREVentYStaSet3_enum) -> bus_creator/860
  outpmodule/1175(VOUTP_FDCVMCDrInpTqBstGn_pct) -> bus_creator/1175
  outpmodule/149(VOUTP_IVIScreen_enum) -> bus_creator/149
  outpmodule/339(VOUTP_HMIKey1FuncSta_enum) -> bus_creator/339
  outpmodule/714(VOUTP_FDSOV2Cmd_flg) -> bus_creator/714
  outpmodule/79(VOUTP_LFPulseCount_enum) -> bus_creator/79
  bus_selector3/44 -> outpmodule/222(VBCM_FrWiperH_flg)  "<VBCM_FrWiperH_flg>"
  bus_selector4/96 -> outpmodule/453(VDDM_ISAMalfuncDetDTC_raw32)  "<VDDM_ISAMalfuncDetDTC_raw32>"
  bus_selector3/175 -> outpmodule/353(VBCM_CLWinLockDrStaMem_enum)  "<VBCM_CLWinLockDrStaMem_enum>"
  outpmodule/338(VOUTP_AutoUnlockMem_enum) -> bus_creator/338
  bus_selector17/39 -> outpmodule/1098(VVMC_ACCObjRelSpd_mps)  "<VVMC_ACCObjRelSpd_mps>"
  bus_selector12/38 -> outpmodule/749(VTHC_ACSubMode_enum)  "<VTHC_ACSubMode_enum>"
  bus_selector11/31 -> outpmodule/699(VSYS_FdcSlpReqRisingEdge_flg)  "<VSYS_FdcSlpReqRisingEdge_flg>"
  bus_selector3/3 -> outpmodule/181(VBCM_HornCtrl_flg)  "<VBCM_HornCtrl_flg>"
  bus_selector4/78 -> outpmodule/435(VDDM_FCM2CSErrDTC_raw32)  "<VDDM_FCM2CSErrDTC_raw32>"
  outpmodule/1054(VOUTP_ReqV2LIVIPopup_enum) -> bus_creator/1054
  bus_selector12/20 -> outpmodule/731(VTHC_BatteryMode_enum)  "<VTHC_BatteryMode_enum>"
  bus_selector11/34 -> outpmodule/702(VSYS_WisrBootReason_raw32)  "<VSYS_WisrBootReason_raw32>"
  outpmodule/1143(VOUTP_FCMLDWRequest_enum) -> bus_creator/1143
  bus_selector3/10 -> outpmodule/188(VBCM_PsDoorSW_flg)  "<VBCM_PsDoorSW_flg>"
  bus_selector14/9 -> outpmodule/993(VTQD_FrActvDmpDisabReq_flg)  "<VTQD_FrActvDmpDisabReq_flg>"
  outpmodule/337(VOUTP_AutoUnlockSta_flg) -> bus_creator/337
  outpmodule/336(VOUTP_AutoLockMem_enum) -> bus_creator/336
  bus_selector4/84 -> outpmodule/441(VDDM_FCM5NoComDTC_raw32)  "<VDDM_FCM5NoComDTC_raw32>"
  outpmodule/770(VOUTP_FDCTHCCREVentZSta_enum) -> bus_creator/770
  bus_selector12/140 -> outpmodule/851(VTHC_FDCTHCLEVentYStaSet7_enum)  "<VTHC_FDCTHCLEVentYStaSet7_enum>"
  outpmodule/284(VOUTP_AmbBrightnessSta1_enum) -> bus_creator/284
  bus_selector11/36 -> outpmodule/704(VSYS_CurrentNmState_enum)  "<VSYS_CurrentNmState_enum>"
  bus_selector17/51 -> outpmodule/1110(VVMC_LeftTurnLightReq_flg)  "<VVMC_LeftTurnLightReq_flg>"
  bus_selector4/14 -> outpmodule/371(VDDM_C1ABM1CSDTC_raw32)  "<VDDM_C1ABM1CSDTC_raw32>"
  bus_selector14/2 -> outpmodule/986(VTQD_TqSourceFr_enum)  "<VTQD_TqSourceFr_enum>"
  bus_selector11/24 -> outpmodule/692(VSYS_SHA3_cnt)  "<VSYS_SHA3_cnt>"
  bus_selector3/45 -> outpmodule/223(VBCM_RrWiper_flg)  "<VBCM_RrWiper_flg>"
  bus_selector3/113 -> outpmodule/291(VBCM_DimSwSta_flg)  "<VBCM_DimSwSta_flg>"
  outpmodule/931(VOUTP_S3ID_raw32) -> bus_creator/931
  outpmodule/332(VOUTP_ACCLevelMem57_enum) -> bus_creator/332
  outpmodule/370(VOUTP_C1ABM1RCDTC_raw32) -> bus_creator/370
  bus_selector4/56 -> outpmodule/413(VDDM_ESC1NoComDTC_raw32)  "<VDDM_ESC1NoComDTC_raw32>"
  outpmodule/652(VOUTP_FDADC12VDetAvg_mV) -> bus_creator/652
  bus_selector3/46 -> outpmodule/224(VBCM_WasherCtrl_enum)  "<VBCM_WasherCtrl_enum>"
  bus_selector2/97 -> outpmodule/100(VAPM_SASCALTimeOut_flg)  "<VAPM_SASCALTimeOut_flg>"
  bus_selector6/12 -> outpmodule/537(VDID_IPSAL_sec)  "<VDID_IPSAL_sec>"
  outpmodule/295(VOUTP_TurnSwSta_enum) -> bus_creator/295
  bus_selector10/21 -> outpmodule/641(VPMM_PwrUpReq_enum)  "<VPMM_PwrUpReq_enum>"
  outpmodule/333(VOUTP_LRightStaCmd_flg) -> bus_creator/333
  outpmodule/1090(VOUTP_LKATOIAct_enum) -> bus_creator/1090
  outpmodule/328(VOUTP_SenstivityPosnCmd_enum) -> bus_creator/328
  outpmodule/327(VOUTP_PTGOpenHeight57_enum) -> bus_creator/327
  outpmodule/736(VOUTP_CCUACMaxLampSts_flg) -> bus_creator/736
  bus_selector4/86 -> outpmodule/443(VDDM_ZoneSCPNoComDTC_raw32)  "<VDDM_ZoneSCPNoComDTC_raw32>"
  bus_selector12/1 -> outpmodule/712(VTHC_FDCompCmd_rpm)  "<VTHC_FDCompCmd_rpm>"
  bus_selector7/28 -> outpmodule/582(VDKC_CalDistance_enum)  "<VDKC_CalDistance_enum>"
  outpmodule/331(VOUTP_ACCLevelMem34_enum) -> bus_creator/331
  bus_selector14/54 -> outpmodule/1038(VTQD_SetSpdLimWarn_flg)  "<VTQD_SetSpdLimWarn_flg>"
  outpmodule/326(VOUTP_PTGOpenHeight34_enum) -> bus_creator/326
  bus_selector11/16 -> outpmodule/684(VSYS_Country2_cnt)  "<VSYS_Country2_cnt>"
  bus_selector12/160 -> outpmodule/871(VTHC_SettempZon1Set2_enum)  "<VTHC_SettempZon1Set2_enum>"
  outpmodule/632(VOUTP_HVPwrSta_flg) -> bus_creator/632
  bus_selector3/125 -> outpmodule/303(VBCM_FDRHandleLampCmd_flg)  "<VBCM_FDRHandleLampCmd_flg>"
  outpmodule/329(VOUTP_TimeGapLevelSta_enum) -> bus_creator/329
  outpmodule/635(VOUTP_RrMCUEnaReq_flg) -> bus_creator/635
  outpmodule/289(VOUTP_AmbBrightnessSta7_enum) -> bus_creator/289
  bus_selector11/25 -> outpmodule/693(VSYS_SHA4_cnt)  "<VSYS_SHA4_cnt>"
  bus_selector4/128 -> outpmodule/485(VDDM_5vAPS1PwrErrDTC_raw32)  "<VDDM_5vAPS1PwrErrDTC_raw32>"
  bus_selector2/56 -> outpmodule/59(VAPM_LRRawWhlSpeedV_flg)  "<VAPM_LRRawWhlSpeedV_flg>"
  bus_selector7/23 -> outpmodule/577(VDKC_FDCSPTGOpen_flg)  "<VDKC_FDCSPTGOpen_flg>"
  outpmodule/325(VOUTP_PTGOpenHeight12_enum) -> bus_creator/325
  outpmodule/343(VOUTP_HMIKey5FuncSta_enum) -> bus_creator/343
  BTHC_outputs/1 -> bus_selector12/1
  outpmodule/555(VOUTP_DKCTimeSN_cnt) -> bus_creator/555
  bus_selector11/27 -> outpmodule/695(VSYS_SHA6_cnt)  "<VSYS_SHA6_cnt>"
  bus_selector4/75 -> outpmodule/432(VDDM_RLRUSSDTC_raw32)  "<VDDM_RLRUSSDTC_raw32>"
  bus_selector3/64 -> outpmodule/242(VBCM_AmbLightColor5_enum)  "<VBCM_AmbLightColor5_enum>"
  outpmodule/322(VOUTP_PTGUserHeight4_cnt) -> bus_creator/322
  bus_selector12/144 -> outpmodule/855(VTHC_FDCTHCCLEVentYStaSet4_enum)  "<VTHC_FDCTHCCLEVentYStaSet4_enum>"
  outpmodule/747(VOUTP_sigAmbAirT_C) -> bus_creator/747
  outpmodule/1018(VOUTP_RrIdcMax_A) -> bus_creator/1018
  outpmodule/197(VOUTP_CTDLockSW_flg) -> bus_creator/197
  bus_selector3/172 -> outpmodule/350(VBCM_DrRWdwReqAP_enum)  "<VBCM_DrRWdwReqAP_enum>"
  bus_selector11/37 -> outpmodule/705(VSYS_ECUGen1_cnt)  "<VSYS_ECUGen1_cnt>"
  bus_selector4/28 -> outpmodule/385(VDDM_BMSRdyDTC_raw32)  "<VDDM_BMSRdyDTC_raw32>"
  bus_selector14/27 -> outpmodule/1011(VTQD_FrRgnPermSta_flg)  "<VTQD_FrRgnPermSta_flg>"
  outpmodule/323(VOUTP_PTGUserHeight5_cnt) -> bus_creator/323
  outpmodule/243(VOUTP_AmbLightColor6_enum) -> bus_creator/243
  bus_selector4/58 -> outpmodule/415(VDDM_EnterNewOperCyc_flg)  "<VDDM_EnterNewOperCyc_flg>"
  bus_selector14/4 -> outpmodule/988(VTQD_FrEDUAvailBrkRgnTq_Nm)  "<VTQD_FrEDUAvailBrkRgnTq_Nm>"
  bus_selector11/7 -> outpmodule/675(VSYS_ECU1_cnt)  "<VSYS_ECU1_cnt>"
  outpmodule/324(VOUTP_PTGUserHeight7_cnt) -> bus_creator/324
  outpmodule/321(VOUTP_PTGUserHeight3_cnt) -> bus_creator/321
  outpmodule/513(VOUTP_FrMCU4PreDTC_raw32) -> bus_creator/513
  bus_selector11/14 -> outpmodule/682(VSYS_Patch2_cnt)  "<VSYS_Patch2_cnt>"
  outpmodule/335(VOUTP_AutoLockSta_flg) -> bus_creator/335
  bus_selector3/66 -> outpmodule/244(VBCM_LampPwr_flg)  "<VBCM_LampPwr_flg>"
  bus_selector12/111 -> outpmodule/822(VTHC_FDCTHCLEVentZStaSet1_enum)  "<VTHC_FDCTHCLEVentZStaSet1_enum>"
  bus_selector14/3 -> outpmodule/987(VTQD_TqSourceRr_enum)  "<VTQD_TqSourceRr_enum>"
  bus_selector8/1 -> outpmodule/605(VDSC_DISCTurn_flg)  "<VDSC_DISCTurn_flg>"
  outpmodule/319(VOUTP_PTGUserHeight1_cnt) -> bus_creator/319
  bus_selector14/25 -> outpmodule/1009(VTQD_RgnAbnorSta_flg)  "<VTQD_RgnAbnorSta_flg>"
  bus_selector11/32 -> outpmodule/700(VSYS_FdcSlpTime_sec)  "<VSYS_FdcSlpTime_sec>"
  bus_selector13/54 -> outpmodule/941(VTPM_RRP20_raw8)  "<VTPM_RRP20_raw8>"
  outpmodule/517(VOUTP_ActAPSPosn_pct) -> bus_creator/517
  outpmodule/271(VOUTP_UserNow_enum) -> bus_creator/271
  bus_selector7/11 -> outpmodule/565(VDKC_KeyAreaPS_enum)  "<VDKC_KeyAreaPS_enum>"
  outpmodule/380(VOUTP_ONtoRdyDTC_raw32) -> bus_creator/380
  outpmodule/240(VOUTP_AmbLightColor3_enum) -> bus_creator/240
  outpmodule/222(VOUTP_FrWiperH_flg) -> bus_creator/222
  outpmodule/320(VOUTP_PTGUserHeight2_cnt) -> bus_creator/320
  bus_selector4/51 -> outpmodule/408(VDDM_APSCorrErrDTC_raw32)  "<VDDM_APSCorrErrDTC_raw32>"
  outpmodule/543(VOUTP_CDEODTR_km) -> bus_creator/543
  bus_selector11/33 -> outpmodule/701(VSYS_PmicBootReason_enum)  "<VSYS_PmicBootReason_enum>"
  bus_selector2/62 -> outpmodule/65(VAPM_RFWhlRotDir_enum)  "<VAPM_RFWhlRotDir_enum>"
  bus_selector16/6 -> outpmodule/1058(VV2L_HVPO120VGrpALDSt_enum)  "<VV2L_HVPO120VGrpALDSt_enum>"
  bus_selector3/168 -> outpmodule/346(VBCM_HMIKey8FuncSta_enum)  "<VBCM_HMIKey8FuncSta_enum>"
  outpmodule/101(VOUTP_SASV_flg) -> bus_creator/101
  bus_selector14/40 -> outpmodule/1024(VTQD_RDCActive_enum)  "<VTQD_RDCActive_enum>"
  outpmodule/1114(VOUTP_ACCObjDstLvl_enum) -> bus_creator/1114
  bus_selector3/50 -> outpmodule/228(VBCM_AmbLightBreath3_enum)  "<VBCM_AmbLightBreath3_enum>"
  bus_selector14/8 -> outpmodule/992(VTQD_PButtonSta_enum)  "<VTQD_PButtonSta_enum>"
  bus_selector3/51 -> outpmodule/229(VBCM_AmbLightBreath4_enum)  "<VBCM_AmbLightBreath4_enum>"
  outpmodule/207(VOUTP_RDRL_flg) -> bus_creator/207
  bus_selector14/7 -> outpmodule/991(VTQD_ShiftGearPosn_enum)  "<VTQD_ShiftGearPosn_enum>"
  bus_selector17/20 -> outpmodule/1079(VVMC_ISOAccLimit_mps2)  "<VVMC_ISOAccLimit_mps2>"
  bus_selector12/30 -> outpmodule/741(VTHC_sigSetTempZon1St_C)  "<VTHC_sigSetTempZon1St_C>"
  outpmodule/439(VOUTP_FCM4NoComDTC_raw32) -> bus_creator/439
  bus_selector2/74 -> outpmodule/77(VAPM_RRPulseCountV_flg)  "<VAPM_RRPulseCountV_flg>"
  outpmodule/619(VOUTP_SysNMmSta_enum) -> bus_creator/619
  outpmodule/318(VOUTP_UserHeightSet_cnt) -> bus_creator/318
  outpmodule/359(VOUTP_C3BMS6CSDTC_raw32) -> bus_creator/359
  outpmodule/330(VOUTP_ACCLevelMem12_enum) -> bus_creator/330
  bus_selector13/90 -> outpmodule/977(VTPM_FlashS4ID_raw)  "<VTPM_FlashS4ID_raw>"
  bus_selector12/21 -> outpmodule/732(VTHC_EDriveMode_enum)  "<VTHC_EDriveMode_enum>"
  outpmodule/334(VOUTP_LLeftStaCmd_flg) -> bus_creator/334
  outpmodule/340(VOUTP_HMIKey2FuncSta_enum) -> bus_creator/340
  bus_selector12/157 -> outpmodule/868(VTHC_FDCTHCCREVentYStaSet5_enum)  "<VTHC_FDCTHCCREVentYStaSet5_enum>"
  bus_selector17/75 -> outpmodule/1134(VVMC_LVDAWarning_flg)  "<VVMC_LVDAWarning_flg>"
